simulink library "outp"  (R2021b)
(part 10 of 10)

  VTPM_LRWheelDebug_flg/1 -> VTPM_LRWheelDebug_flg_Inproc/1  "VTPM_LRWheelDebug_flg"
  VTPM_LRWheelDebug_flg_Inproc/1 -> UnitConverter666/1
  UnitConverter666/1 -> VOUTP_LRWheelDebug_flg/1  "VOUTP_LRWheelDebug_flg"
  VTPM_RFWheelDebug_flg/1 -> VTPM_RFWheelDebug_flg_Inproc/1  "VTPM_RFWheelDebug_flg"
  VTPM_RFWheelDebug_flg_Inproc/1 -> UnitConverter667/1
  UnitConverter667/1 -> VOUTP_RFWheelDebug_flg/1  "VOUTP_RFWheelDebug_flg"
  VTPM_RRWheelDebug_flg/1 -> VTPM_RRWheelDebug_flg_Inproc/1  "VTPM_RRWheelDebug_flg"
  VTPM_RRWheelDebug_flg_Inproc/1 -> UnitConverter668/1
  UnitConverter668/1 -> VOUTP_RRWheelDebug_flg/1  "VOUTP_RRWheelDebug_flg"
  VTPM_TPMSResButtAllow_flg/1 -> VTPM_TPMSResButtAllow_flg_Inproc/1  "VTPM_TPMSResButtAllow_flg"
  VTPM_TPMSResButtAllow_flg_Inproc/1 -> UnitConverter669/1
  UnitConverter669/1 -> VOUTP_TPMSResButtAllow_flg/1  "VOUTP_TPMSResButtAllow_flg"
  VTPM_TPMSCaliButtAllow_flg/1 -> VTPM_TPMSCaliButtAllow_flg_Inproc/1  "VTPM_TPMSCaliButtAllow_flg"
  VTPM_TPMSCaliButtAllow_flg_Inproc/1 -> UnitConverter670/1
  UnitConverter670/1 -> VOUTP_TPMSCaliButtAllow_flg/1  "VOUTP_TPMSCaliButtAllow_flg"
  VTPM_LFPressIndi_enum/1 -> VTPM_LFPressIndi_enum_Inproc/1  "VTPM_LFPressIndi_enum"
  VTPM_LFPressIndi_enum_Inproc/1 -> UnitConverter671/1
  UnitConverter671/1 -> VOUTP_LFPressIndi_enum/1  "VOUTP_LFPressIndi_enum"
  VTPM_RFPressIndi_enum/1 -> VTPM_RFPressIndi_enum_Inproc/1  "VTPM_RFPressIndi_enum"
  VTPM_RFPressIndi_enum_Inproc/1 -> UnitConverter672/1
  UnitConverter672/1 -> VOUTP_RFPressIndi_enum/1  "VOUTP_RFPressIndi_enum"
  VTPM_LRPressIndi_enum/1 -> VTPM_LRPressIndi_enum_Inproc/1  "VTPM_LRPressIndi_enum"
  VTPM_LRPressIndi_enum_Inproc/1 -> UnitConverter673/1
  UnitConverter673/1 -> VOUTP_LRPressIndi_enum/1  "VOUTP_LRPressIndi_enum"
  VTPM_RRPressIndi_enum/1 -> VTPM_RRPressIndi_enum_Inproc/1  "VTPM_RRPressIndi_enum"
  VTPM_RRPressIndi_enum_Inproc/1 -> UnitConverter674/1
  UnitConverter674/1 -> VOUTP_RRPressIndi_enum/1  "VOUTP_RRPressIndi_enum"
  VTPM_TPMSWarnIndi_enum/1 -> VTPM_TPMSWarnIndi_enum_Inproc/1  "VTPM_TPMSWarnIndi_enum"
  VTPM_TPMSWarnIndi_enum_Inproc/1 -> UnitConverter675/1
  UnitConverter675/1 -> VOUTP_TPMSWarnIndi_enum/1  "VOUTP_TPMSWarnIndi_enum"
  VTPM_LFWheelTmpIndi_flg/1 -> VTPM_LFWheelTmpIndi_flg_Inproc/1  "VTPM_LFWheelTmpIndi_flg"
  VTPM_LFWheelTmpIndi_flg_Inproc/1 -> UnitConverter676/1
  UnitConverter676/1 -> VOUTP_LFWheelTmpIndi_flg/1  "VOUTP_LFWheelTmpIndi_flg"
  VTPM_RFWheelTmpIndi_flg/1 -> VTPM_RFWheelTmpIndi_flg_Inproc/1  "VTPM_RFWheelTmpIndi_flg"
  VTPM_RFWheelTmpIndi_flg_Inproc/1 -> UnitConverter677/1
  UnitConverter677/1 -> VOUTP_RFWheelTmpIndi_flg/1  "VOUTP_RFWheelTmpIndi_flg"
  VTPM_LRWheelTmpIndi_flg/1 -> VTPM_LRWheelTmpIndi_flg_Inproc/1  "VTPM_LRWheelTmpIndi_flg"
  VTPM_LRWheelTmpIndi_flg_Inproc/1 -> UnitConverter678/1
  UnitConverter678/1 -> VOUTP_LRWheelTmpIndi_flg/1  "VOUTP_LRWheelTmpIndi_flg"
  VTPM_RRWheelTmpIndi_flg/1 -> VTPM_RRWheelTmpIndi_flg_Inproc/1  "VTPM_RRWheelTmpIndi_flg"
  VTPM_RRWheelTmpIndi_flg_Inproc/1 -> UnitConverter679/1
  UnitConverter679/1 -> VOUTP_RRWheelTmpIndi_flg/1  "VOUTP_RRWheelTmpIndi_flg"
  VTPM_LFWheelPSW_raw8/1 -> VTPM_LFWheelPSW_raw8_Inproc/1  "VTPM_LFWheelPSW_raw8"
  VTPM_LFWheelPSW_raw8_Inproc/1 -> UnitConverter680/1
  UnitConverter680/1 -> VOUTP_LFWheelPSW_raw8/1  "VOUTP_LFWheelPSW_raw8"
  VTPM_LRWheelPSW_raw8/1 -> VTPM_LRWheelPSW_raw8_Inproc/1  "VTPM_LRWheelPSW_raw8"
  VTPM_LRWheelPSW_raw8_Inproc/1 -> UnitConverter681/1
  UnitConverter681/1 -> VOUTP_LRWheelPSW_raw8/1  "VOUTP_LRWheelPSW_raw8"
  VTPM_RFWheelPSW_raw8/1 -> VTPM_RFWheelPSW_raw8_Inproc/1  "VTPM_RFWheelPSW_raw8"
  VTPM_RFWheelPSW_raw8_Inproc/1 -> UnitConverter682/1
  UnitConverter682/1 -> VOUTP_RFWheelPSW_raw8/1  "VOUTP_RFWheelPSW_raw8"
  VTPM_RRWheelPSW_raw8/1 -> VTPM_RRWheelPSW_raw8_Inproc/1  "VTPM_RRWheelPSW_raw8"
  VTPM_RRWheelPSW_raw8_Inproc/1 -> UnitConverter683/1
  UnitConverter683/1 -> VOUTP_RRWheelPSW_raw8/1  "VOUTP_RRWheelPSW_raw8"
  VTPM_CWheelTips_enum/1 -> VTPM_CWheelTips_enum_Inproc/1  "VTPM_CWheelTips_enum"
  VTPM_CWheelTips_enum_Inproc/1 -> UnitConverter684/1
  UnitConverter684/1 -> VOUTP_CWheelTips_enum/1  "VOUTP_CWheelTips_enum"
  VTPM_AutoLTips_enum/1 -> VTPM_AutoLTips_enum_Inproc/1  "VTPM_AutoLTips_enum"
  VTPM_AutoLTips_enum_Inproc/1 -> UnitConverter685/1
  UnitConverter685/1 -> VOUTP_AutoLTips_enum/1  "VOUTP_AutoLTips_enum"
  VTPM_LFSensorMode_flg/1 -> VTPM_LFSensorMode_flg_Inproc/1  "VTPM_LFSensorMode_flg"
  VTPM_LFSensorMode_flg_Inproc/1 -> UnitConverter686/1
  UnitConverter686/1 -> VOUTP_LFSensorMode_flg/1  "VOUTP_LFSensorMode_flg"
  VTPM_RFSensorMode_flg/1 -> VTPM_RFSensorMode_flg_Inproc/1  "VTPM_RFSensorMode_flg"
  VTPM_RFSensorMode_flg_Inproc/1 -> UnitConverter687/1
  UnitConverter687/1 -> VOUTP_RFSensorMode_flg/1  "VOUTP_RFSensorMode_flg"
  VTPM_LRSensorMode_flg/1 -> VTPM_LRSensorMode_flg_Inproc/1  "VTPM_LRSensorMode_flg"
  VTPM_LRSensorMode_flg_Inproc/1 -> UnitConverter688/1
  UnitConverter688/1 -> VOUTP_LRSensorMode_flg/1  "VOUTP_LRSensorMode_flg"
  VTPM_RRSensorMode_flg/1 -> VTPM_RRSensorMode_flg_Inproc/1  "VTPM_RRSensorMode_flg"
  VTPM_RRSensorMode_flg_Inproc/1 -> UnitConverter689/1
  UnitConverter689/1 -> VOUTP_RRSensorMode_flg/1  "VOUTP_RRSensorMode_flg"
  VTPM_S1ID_raw32/1 -> VTPM_S1ID_raw32_Inproc/1  "VTPM_S1ID_raw32"
  VTPM_S1ID_raw32_Inproc/1 -> UnitConverter690/1
  UnitConverter690/1 -> VOUTP_S1ID_raw32/1  "VOUTP_S1ID_raw32"
  VTPM_S2ID_raw32/1 -> VTPM_S2ID_raw32_Inproc/1  "VTPM_S2ID_raw32"
  VTPM_S2ID_raw32_Inproc/1 -> UnitConverter691/1
  UnitConverter691/1 -> VOUTP_S2ID_raw32/1  "VOUTP_S2ID_raw32"
  VTPM_S3ID_raw32/1 -> VTPM_S3ID_raw32_Inproc/1  "VTPM_S3ID_raw32"
  VTPM_S3ID_raw32_Inproc/1 -> UnitConverter692/1
  UnitConverter692/1 -> VOUTP_S3ID_raw32/1  "VOUTP_S3ID_raw32"
  VTPM_S4ID_raw32/1 -> VTPM_S4ID_raw32_Inproc/1  "VTPM_S4ID_raw32"
  VTPM_S4ID_raw32_Inproc/1 -> UnitConverter693/1
  UnitConverter693/1 -> VOUTP_S4ID_raw32/1  "VOUTP_S4ID_raw32"
  VTPM_S1L_enum/1 -> VTPM_S1L_enum_Inproc/1  "VTPM_S1L_enum"
  VTPM_S1L_enum_Inproc/1 -> UnitConverter694/1
  UnitConverter694/1 -> VOUTP_S1L_enum/1  "VOUTP_S1L_enum"
  VTPM_S2L_enum/1 -> VTPM_S2L_enum_Inproc/1  "VTPM_S2L_enum"
  VTPM_S2L_enum_Inproc/1 -> UnitConverter695/1
  UnitConverter695/1 -> VOUTP_S2L_enum/1  "VOUTP_S2L_enum"
  VTPM_S3L_enum/1 -> VTPM_S3L_enum_Inproc/1  "VTPM_S3L_enum"
  VTPM_S3L_enum_Inproc/1 -> UnitConverter696/1
  UnitConverter696/1 -> VOUTP_S3L_enum/1  "VOUTP_S3L_enum"
  VTPM_S4L_enum/1 -> VTPM_S4L_enum_Inproc/1  "VTPM_S4L_enum"
  VTPM_S4L_enum_Inproc/1 -> UnitConverter697/1
  UnitConverter697/1 -> VOUTP_S4L_enum/1  "VOUTP_S4L_enum"
  VTPM_ALFin_flg/1 -> VTPM_ALFin_flg_Inproc/1  "VTPM_ALFin_flg"
  VTPM_ALFin_flg_Inproc/1 -> UnitConverter698/1
  UnitConverter698/1 -> VOUTP_ALFin_flg/1  "VOUTP_ALFin_flg"
  VTPM_LFP20_raw8/1 -> VTPM_LFP20_raw8_Inproc/1  "VTPM_LFP20_raw8"
  VTPM_LFP20_raw8_Inproc/1 -> UnitConverter699/1
  UnitConverter699/1 -> VOUTP_LFP20_raw8/1  "VOUTP_LFP20_raw8"
  VTPM_RFP20_raw8/1 -> VTPM_RFP20_raw8_Inproc/1  "VTPM_RFP20_raw8"
  VTPM_RFP20_raw8_Inproc/1 -> UnitConverter700/1
  UnitConverter700/1 -> VOUTP_RFP20_raw8/1  "VOUTP_RFP20_raw8"
  VTPM_LRP20_raw8/1 -> VTPM_LRP20_raw8_Inproc/1  "VTPM_LRP20_raw8"
  VTPM_LRP20_raw8_Inproc/1 -> UnitConverter701/1
  UnitConverter701/1 -> VOUTP_LRP20_raw8/1  "VOUTP_LRP20_raw8"
  VTPM_RRP20_raw8/1 -> VTPM_RRP20_raw8_Inproc/1  "VTPM_RRP20_raw8"
  VTPM_RRP20_raw8_Inproc/1 -> UnitConverter702/1
  UnitConverter702/1 -> VOUTP_RRP20_raw8/1  "VOUTP_RRP20_raw8"
  VTPM_FAT_flg/1 -> VTPM_FAT_flg_Inproc/1  "VTPM_FAT_flg"
  VTPM_FAT_flg_Inproc/1 -> UnitConverter703/1
  UnitConverter703/1 -> VOUTP_FAT_flg/1  "VOUTP_FAT_flg"
  VTPM_IDin_raw32/1 -> VTPM_IDin_raw32_Inproc/1  "VTPM_IDin_raw32"
  VTPM_IDin_raw32_Inproc/1 -> UnitConverter704/1
  UnitConverter704/1 -> VOUTP_IDin_raw32/1  "VOUTP_IDin_raw32"
  VTPM_S1WheelDebugALTU_pct/1 -> VTPM_S1WheelDebugALTU_pct_Inproc/1  "VTPM_S1WheelDebugALTU_pct"
  VTPM_S1WheelDebugALTU_pct_Inproc/1 -> UnitConverter705/1
  UnitConverter705/1 -> VOUTP_S1WheelDebugALTU_pct/1  "VOUTP_S1WheelDebugALTU_pct"
  VTPM_S2WheelDebugALTU_pct/1 -> VTPM_S2WheelDebugALTU_pct_Inproc/1  "VTPM_S2WheelDebugALTU_pct"
  VTPM_S2WheelDebugALTU_pct_Inproc/1 -> UnitConverter706/1
  UnitConverter706/1 -> VOUTP_S2WheelDebugALTU_pct/1  "VOUTP_S2WheelDebugALTU_pct"
  VTPM_S3WheelDebugALTU_pct/1 -> VTPM_S3WheelDebugALTU_pct_Inproc/1  "VTPM_S3WheelDebugALTU_pct"
  VTPM_S3WheelDebugALTU_pct_Inproc/1 -> UnitConverter707/1
  UnitConverter707/1 -> VOUTP_S3WheelDebugALTU_pct/1  "VOUTP_S3WheelDebugALTU_pct"
  VTPM_S4WheelDebugALTU_pct/1 -> VTPM_S4WheelDebugALTU_pct_Inproc/1  "VTPM_S4WheelDebugALTU_pct"
  VTPM_S4WheelDebugALTU_pct_Inproc/1 -> UnitConverter708/1
  UnitConverter708/1 -> VOUTP_S4WheelDebugALTU_pct/1  "VOUTP_S4WheelDebugALTU_pct"
  VTPM_ID1messageALTU_raw8/1 -> VTPM_ID1messageALTU_raw8_Inproc/1  "VTPM_ID1messageALTU_raw8"
  VTPM_ID1messageALTU_raw8_Inproc/1 -> UnitConverter709/1
  UnitConverter709/1 -> VOUTP_ID1messageALTU_raw8/1  "VOUTP_ID1messageALTU_raw8"
  VTPM_ID2messageALTU_raw8/1 -> VTPM_ID2messageALTU_raw8_Inproc/1  "VTPM_ID2messageALTU_raw8"
  VTPM_ID2messageALTU_raw8_Inproc/1 -> UnitConverter710/1
  UnitConverter710/1 -> VOUTP_ID2messageALTU_raw8/1  "VOUTP_ID2messageALTU_raw8"
  VTPM_ID3messageALTU_raw8/1 -> VTPM_ID3messageALTU_raw8_Inproc/1  "VTPM_ID3messageALTU_raw8"
  VTPM_ID3messageALTU_raw8_Inproc/1 -> UnitConverter711/1
  UnitConverter711/1 -> VOUTP_ID3messageALTU_raw8/1  "VOUTP_ID3messageALTU_raw8"
  VTPM_ID4messageALTU_raw8/1 -> VTPM_ID4messageALTU_raw8_Inproc/1  "VTPM_ID4messageALTU_raw8"
  VTPM_ID4messageALTU_raw8_Inproc/1 -> UnitConverter712/1
  UnitConverter712/1 -> VOUTP_ID4messageALTU_raw8/1  "VOUTP_ID4messageALTU_raw8"
  VTPM_Chkfin_flg/1 -> VTPM_Chkfin_flg_Inproc/1  "VTPM_Chkfin_flg"
  VTPM_Chkfin_flg_Inproc/1 -> UnitConverter713/1
  UnitConverter713/1 -> VOUTP_Chkfin_flg/1  "VOUTP_Chkfin_flg"
  VTPM_SetIDLoc_flg/1 -> VTPM_SetIDLoc_flg_Inproc/1  "VTPM_SetIDLoc_flg"
  VTPM_SetIDLoc_flg_Inproc/1 -> UnitConverter714/1
  UnitConverter714/1 -> VOUTP_SetIDLoc_flg/1  "VOUTP_SetIDLoc_flg"
  VTPM_TPMSStorge_flg/1 -> VTPM_TPMSStorge_flg_Inproc/1  "VTPM_TPMSStorge_flg"
  VTPM_TPMSStorge_flg_Inproc/1 -> UnitConverter715/1
  UnitConverter715/1 -> VOUTP_TPMSStorge_flg/1  "VOUTP_TPMSStorge_flg"
  VTPM_ChkStorge_flg/1 -> VTPM_ChkStorge_flg_Inproc/1  "VTPM_ChkStorge_flg"
  VTPM_ChkStorge_flg_Inproc/1 -> UnitConverter716/1
  UnitConverter716/1 -> VOUTP_ChkStorge_flg/1  "VOUTP_ChkStorge_flg"
  VTPM_TPMSResButt_flg/1 -> VTPM_TPMSResButt_flg_Inproc/1  "VTPM_TPMSResButt_flg"
  VTPM_TPMSResButt_flg_Inproc/1 -> UnitConverter717/1
  UnitConverter717/1 -> VOUTP_TPMSResButt_flg/1  "VOUTP_TPMSResButt_flg"
  VTPM_LFPindi_enum/1 -> VTPM_LFPindi_enum_Inproc/1  "VTPM_LFPindi_enum"
  VTPM_LFPindi_enum_Inproc/1 -> UnitConverter718/1
  UnitConverter718/1 -> VOUTP_LFPindi_enum/1  "VOUTP_LFPindi_enum"
  VTPM_RFPind_enum/1 -> VTPM_RFPind_enum_Inproc/1  "VTPM_RFPind_enum"
  VTPM_RFPind_enum_Inproc/1 -> UnitConverter719/1
  UnitConverter719/1 -> VOUTP_RFPind_enum/1  "VOUTP_RFPind_enum"
  VTPM_LRPindi_enum/1 -> VTPM_LRPindi_enum_Inproc/1  "VTPM_LRPindi_enum"
  VTPM_LRPindi_enum_Inproc/1 -> UnitConverter720/1
  UnitConverter720/1 -> VOUTP_LRPindi_enum/1  "VOUTP_LRPindi_enum"
  VTPM_RRPindi_enum/1 -> VTPM_RRPindi_enum_Inproc/1  "VTPM_RRPindi_enum"
  VTPM_RRPindi_enum_Inproc/1 -> UnitConverter721/1
  UnitConverter721/1 -> VOUTP_RRPindi_enum/1  "VOUTP_RRPindi_enum"
  VTPM_WriteChkLFID_raw/1 -> VTPM_WriteChkLFID_raw_Inproc/1  "VTPM_WriteChkLFID_raw"
  VTPM_WriteChkLFID_raw_Inproc/1 -> UnitConverter722/1
  UnitConverter722/1 -> VOUTP_WriteChkLFID_raw/1  "VOUTP_WriteChkLFID_raw"
  VTPM_WriteChkRFID_raw/1 -> VTPM_WriteChkRFID_raw_Inproc/1  "VTPM_WriteChkRFID_raw"
  VTPM_WriteChkRFID_raw_Inproc/1 -> UnitConverter723/1
  UnitConverter723/1 -> VOUTP_WriteChkRFID_raw/1  "VOUTP_WriteChkRFID_raw"
  VTPM_WriteChkLRID_raw/1 -> VTPM_WriteChkLRID_raw_Inproc/1  "VTPM_WriteChkLRID_raw"
  VTPM_WriteChkLRID_raw_Inproc/1 -> UnitConverter724/1
  UnitConverter724/1 -> VOUTP_WriteChkLRID_raw/1  "VOUTP_WriteChkLRID_raw"
  VTPM_WriteChkRRID_raw/1 -> VTPM_WriteChkRRID_raw_Inproc/1  "VTPM_WriteChkRRID_raw"
  VTPM_WriteChkRRID_raw_Inproc/1 -> UnitConverter725/1
  UnitConverter725/1 -> VOUTP_WriteChkRRID_raw/1  "VOUTP_WriteChkRRID_raw"
  VTPM_WriteChkfinLFID_raw/1 -> VTPM_WriteChkfinLFID_raw_Inproc/1  "VTPM_WriteChkfinLFID_raw"
  VTPM_WriteChkfinLFID_raw_Inproc/1 -> UnitConverter726/1
  UnitConverter726/1 -> VOUTP_WriteChkfinLFID_raw/1  "VOUTP_WriteChkfinLFID_raw"
  VTPM_WriteChkfinRFID_raw/1 -> VTPM_WriteChkfinRFID_raw_Inproc/1  "VTPM_WriteChkfinRFID_raw"
  VTPM_WriteChkfinRFID_raw_Inproc/1 -> UnitConverter727/1
  UnitConverter727/1 -> VOUTP_WriteChkfinRFID_raw/1  "VOUTP_WriteChkfinRFID_raw"
  VTPM_WriteChkfinLRID_raw/1 -> VTPM_WriteChkfinLRID_raw_Inproc/1  "VTPM_WriteChkfinLRID_raw"
  VTPM_WriteChkfinLRID_raw_Inproc/1 -> UnitConverter728/1
  UnitConverter728/1 -> VOUTP_WriteChkfinLRID_raw/1  "VOUTP_WriteChkfinLRID_raw"
  VTPM_WriteChkfinRRID_raw/1 -> VTPM_WriteChkfinRRID_raw_Inproc/1  "VTPM_WriteChkfinRRID_raw"
  VTPM_WriteChkfinRRID_raw_Inproc/1 -> UnitConverter729/1
  UnitConverter729/1 -> VOUTP_WriteChkfinRRID_raw/1  "VOUTP_WriteChkfinRRID_raw"
  VTPM_Flashchkdatavalid_enum/1 -> VTPM_Flashchkdatavalid_enum_Inproc/1  "VTPM_Flashchkdatavalid_enum"
  VTPM_Flashchkdatavalid_enum_Inproc/1 -> UnitConverter730/1
  UnitConverter730/1 -> VOUTP_Flashchkdatavalid_enum/1  "VOUTP_Flashchkdatavalid_enum"
  VTPM_Flashdatavalid_enum/1 -> VTPM_Flashdatavalid_enum_Inproc/1  "VTPM_Flashdatavalid_enum"
  VTPM_Flashdatavalid_enum_Inproc/1 -> UnitConverter731/1
  UnitConverter731/1 -> VOUTP_Flashdatavalid_enum/1  "VOUTP_Flashdatavalid_enum"
  VTPM_unlearnSfali_flg/1 -> VTPM_unlearnSfali_flg_Inproc/1  "VTPM_unlearnSfali_flg"
  VTPM_unlearnSfali_flg_Inproc/1 -> UnitConverter732/1
  UnitConverter732/1 -> VOUTP_unlearnSfali_flg/1  "VOUTP_unlearnSfali_flg"
  VTPM_unlearnSfailvalid_enum/1 -> VTPM_unlearnSfailvalid_enum_Inproc/1  "VTPM_unlearnSfailvalid_enum"
  VTPM_unlearnSfailvalid_enum_Inproc/1 -> UnitConverter733/1
  UnitConverter733/1 -> VOUTP_unlearnSfailvalid_enum/1  "VOUTP_unlearnSfailvalid_enum"
  VTPM_Prepresstempvalid_enum/1 -> VTPM_Prepresstempvalid_enum_Inproc/1  "VTPM_Prepresstempvalid_enum"
  VTPM_Prepresstempvalid_enum_Inproc/1 -> UnitConverter734/1
  UnitConverter734/1 -> VOUTP_Prepresstempvalid_enum/1  "VOUTP_Prepresstempvalid_enum"
  VTPM_FlashS1ID_raw/1 -> VTPM_FlashS1ID_raw_Inproc/1  "VTPM_FlashS1ID_raw"
  VTPM_FlashS1ID_raw_Inproc/1 -> UnitConverter735/1
  UnitConverter735/1 -> VOUTP_FlashS1ID_raw/1  "VOUTP_FlashS1ID_raw"
  VTPM_FlashS2ID_raw/1 -> VTPM_FlashS2ID_raw_Inproc/1  "VTPM_FlashS2ID_raw"
  VTPM_FlashS2ID_raw_Inproc/1 -> UnitConverter736/1
  UnitConverter736/1 -> VOUTP_FlashS2ID_raw/1  "VOUTP_FlashS2ID_raw"
  VTPM_FlashS3ID_raw/1 -> VTPM_FlashS3ID_raw_Inproc/1  "VTPM_FlashS3ID_raw"
  VTPM_FlashS3ID_raw_Inproc/1 -> UnitConverter737/1
  UnitConverter737/1 -> VOUTP_FlashS3ID_raw/1  "VOUTP_FlashS3ID_raw"
  VTPM_FlashS4ID_raw/1 -> VTPM_FlashS4ID_raw_Inproc/1  "VTPM_FlashS4ID_raw"
  VTPM_FlashS4ID_raw_Inproc/1 -> UnitConverter738/1
  UnitConverter738/1 -> VOUTP_FlashS4ID_raw/1  "VOUTP_FlashS4ID_raw"
  VTPM_FlashIDvalid_enum/1 -> VTPM_FlashIDvalid_enum_Inproc/1  "VTPM_FlashIDvalid_enum"
  VTPM_FlashIDvalid_enum_Inproc/1 -> UnitConverter739/1
  UnitConverter739/1 -> VOUTP_FlashIDvalid_enum/1  "VOUTP_FlashIDvalid_enum"
  VTPM_WritingCnt_enum/1 -> VTPM_WritingCnt_enum_Inproc/1  "VTPM_WritingCnt_enum"
  VTPM_WritingCnt_enum_Inproc/1 -> UnitConverter740/1
  UnitConverter740/1 -> VOUTP_WritingCnt_enum/1  "VOUTP_WritingCnt_enum"
  VTPM_TPMSTLCmd_flg/1 -> VTPM_TPMSTLCmd_flg_Inproc/1  "VTPM_TPMSTLCmd_flg"
  VTPM_TPMSTLCmd_flg_Inproc/1 -> UnitConverter741/1
  UnitConverter741/1 -> VOUTP_TPMSTLCmd_flg/1  "VOUTP_TPMSTLCmd_flg"
  VTPM_LProgress_enum/1 -> VTPM_LProgress_enum_Inproc/1  "VTPM_LProgress_enum"
  VTPM_LProgress_enum_Inproc/1 -> UnitConverter742/1
  UnitConverter742/1 -> VOUTP_LProgress_enum/1  "VOUTP_LProgress_enum"
  VTPM_TPMSSensorIDRegStart_flg/1 -> VTPM_TPMSSensorIDRegStart_flg_Inproc/1  "VTPM_TPMSSensorIDRegStart_flg"
  VTPM_TPMSSensorIDRegStart_flg_Inproc/1 -> UnitConverter743/1
  UnitConverter743/1 -> VOUTP_TPMSSensorIDRegStart_flg/1  "VOUTP_TPMSSensorIDRegStart_flg"
  VTPM_ModelVersion_raw/1 -> VTPM_ModelVersion_raw_Inproc/1  "VTPM_ModelVersion_raw"
  VTPM_ModelVersion_raw_Inproc/1 -> UnitConverter744/1
  UnitConverter744/1 -> VOUTP_ModelVersion_raw/1  "VOUTP_ModelVersion_raw"
  VTPM_ModelVersionChksum_raw/1 -> VTPM_ModelVersionChksum_raw_Inproc/1  "VTPM_ModelVersionChksum_raw"
  VTPM_ModelVersionChksum_raw_Inproc/1 -> UnitConverter745/1
  UnitConverter745/1 -> VOUTP_ModelVersionChksum_raw/1  "VOUTP_ModelVersionChksum_raw"
  VTQD_VCUMCUCtrlMdTQD_enum/1 -> VTQD_VCUMCUCtrlMdTQD_enum_Inproc/1  "VTQD_VCUMCUCtrlMdTQD_enum"
  VTQD_VCUMCUCtrlMdTQD_enum_Inproc/1 -> UnitConverter746/1
  UnitConverter746/1 -> VOUTP_VCUMCUCtrlMdTQD_enum/1  "VOUTP_VCUMCUCtrlMdTQD_enum"
  VTQD_CreepSpdReq_rpm/1 -> VTQD_CreepSpdReq_rpm_Inproc/1  "VTQD_CreepSpdReq_rpm"
  VTQD_CreepSpdReq_rpm_Inproc/1 -> UnitConverter747/1
  UnitConverter747/1 -> VOUTP_CreepSpdReq_rpm/1  "VOUTP_CreepSpdReq_rpm"
  VTQD_CreepIND_enum/1 -> VTQD_CreepIND_enum_Inproc/1  "VTQD_CreepIND_enum"
  VTQD_CreepIND_enum_Inproc/1 -> UnitConverter748/1
  UnitConverter748/1 -> VOUTP_CreepIND_enum/1  "VOUTP_CreepIND_enum"
  VTQD_ActTUpAIND_enum/1 -> VTQD_ActTUpAIND_enum_Inproc/1  "VTQD_ActTUpAIND_enum"
  VTQD_ActTUpAIND_enum_Inproc/1 -> UnitConverter749/1
  UnitConverter749/1 -> VOUTP_ActTUpAIND_enum/1  "VOUTP_ActTUpAIND_enum"
  VTQD_VCUMCUDemHiPosVal_rpm/1 -> VTQD_VCUMCUDemHiPosVal_rpm_Inproc/1  "VTQD_VCUMCUDemHiPosVal_rpm"
  VTQD_VCUMCUDemHiPosVal_rpm_Inproc/1 -> UnitConverter750/1
  UnitConverter750/1 -> VOUTP_VCUMCUDemHiPosVal_rpm/1  "VOUTP_VCUMCUDemHiPosVal_rpm"
  VTQD_VehAcclLimitTG_mps2/1 -> VTQD_VehAcclLimitTG_mps2_Inproc/1  "VTQD_VehAcclLimitTG_mps2"
  VTQD_VehAcclLimitTG_mps2_Inproc/1 -> UnitConverter751/1
  UnitConverter751/1 -> VOUTP_VehAcclLimitTG_mps2/1  "VOUTP_VehAcclLimitTG_mps2"
  VTQD_VCUEBSHHSw_enum/1 -> VTQD_VCUEBSHHSw_enum_Inproc/1  "VTQD_VCUEBSHHSw_enum"
  VTQD_VCUEBSHHSw_enum_Inproc/1 -> UnitConverter752/1
  UnitConverter752/1 -> VOUTP_VCUEBSHHSw_enum/1  "VOUTP_VCUEBSHHSw_enum"
  VTQD_VCUEBSRd4BR_enum/1 -> VTQD_VCUEBSRd4BR_enum_Inproc/1  "VTQD_VCUEBSRd4BR_enum"
  VTQD_VCUEBSRd4BR_enum_Inproc/1 -> UnitConverter753/1
  UnitConverter753/1 -> VOUTP_VCUEBSRd4BR_enum/1  "VOUTP_VCUEBSRd4BR_enum"
  VTQD_ParkingProtectWarning_flg/1 -> VTQD_ParkingProtectWarning_flg_Inproc/1  "VTQD_ParkingProtectWarning_flg"
  VTQD_ParkingProtectWarning_flg_Inproc/1 -> UnitConverter754/1
  UnitConverter754/1 -> VOUTP_ParkingProtectWarning_flg/1  "VOUTP_ParkingProtectWarning_flg"
  VTQD_ActDriveMode_enum/1 -> VTQD_ActDriveMode_enum_Inproc/1  "VTQD_ActDriveMode_enum"
  VTQD_ActDriveMode_enum_Inproc/1 -> UnitConverter755/1
  UnitConverter755/1 -> VOUTP_ActDriveMode_enum/1  "VOUTP_ActDriveMode_enum"
  VTQD_VCU4PweLmtInd_flg/1 -> VTQD_VCU4PweLmtInd_flg_Inproc/1  "VTQD_VCU4PweLmtInd_flg"
  VTQD_VCU4PweLmtInd_flg_Inproc/1 -> UnitConverter756/1
  UnitConverter756/1 -> VOUTP_VCU4PweLmtInd_flg/1  "VOUTP_VCU4PweLmtInd_flg"
  VTQD_GearFlashIndDis_flg/1 -> VTQD_GearFlashIndDis_flg_Inproc/1  "VTQD_GearFlashIndDis_flg"
  VTQD_GearFlashIndDis_flg_Inproc/1 -> UnitConverter757/1
  UnitConverter757/1 -> VOUTP_GearFlashIndDis_flg/1  "VOUTP_GearFlashIndDis_flg"
  VTQD_GearFlashInd_flg/1 -> VTQD_GearFlashInd_flg_Inproc/1  "VTQD_GearFlashInd_flg"
  VTQD_GearFlashInd_flg_Inproc/1 -> UnitConverter758/1
  UnitConverter758/1 -> VOUTP_GearFlashInd_flg/1  "VOUTP_GearFlashInd_flg"
  VTQD_SpdLimSta_flg/1 -> VTQD_SpdLimSta_flg_Inproc/1  "VTQD_SpdLimSta_flg"
  VTQD_SpdLimSta_flg_Inproc/1 -> UnitConverter759/1
  UnitConverter759/1 -> VOUTP_SpdLimSta_flg/1  "VOUTP_SpdLimSta_flg"
  VTQD_VehSpdLimitTG_kph/1 -> VTQD_VehSpdLimitTG_kph_Inproc/1  "VTQD_VehSpdLimitTG_kph"
  VTQD_VehSpdLimitTG_kph_Inproc/1 -> UnitConverter760/1
  UnitConverter760/1 -> VOUTP_VehSpdLimitTG_kph/1  "VOUTP_VehSpdLimitTG_kph"
  VTQD_VCUTMVehSpd_kph/1 -> VTQD_VCUTMVehSpd_kph_Inproc/1  "VTQD_VCUTMVehSpd_kph"
  VTQD_VCUTMVehSpd_kph_Inproc/1 -> UnitConverter761/1
  UnitConverter761/1 -> VOUTP_VCUTMVehSpd_kph/1  "VOUTP_VCUTMVehSpd_kph"
  VTQD_TMTqReq_Nm/1 -> VTQD_TMTqReq_Nm_Inproc/1  "VTQD_TMTqReq_Nm"
  VTQD_TMTqReq_Nm_Inproc/1 -> UnitConverter762/1
  UnitConverter762/1 -> VOUTP_TMTqReq_Nm/1  "VOUTP_TMTqReq_Nm"
  VTQD_VCUBCMBuzzReq_flg/1 -> VTQD_VCUBCMBuzzReq_flg_Inproc/1  "VTQD_VCUBCMBuzzReq_flg"
  VTQD_VCUBCMBuzzReq_flg_Inproc/1 -> UnitConverter763/1
  UnitConverter763/1 -> VOUTP_VCUBCMBuzzReq_flg/1  "VOUTP_VCUBCMBuzzReq_flg"
  VTQD_VCUEBSHBSw_enum/1 -> VTQD_VCUEBSHBSw_enum_Inproc/1  "VTQD_VCUEBSHBSw_enum"
  VTQD_VCUEBSHBSw_enum_Inproc/1 -> UnitConverter764/1
  UnitConverter764/1 -> VOUTP_VCUEBSHBSw_enum/1  "VOUTP_VCUEBSHBSw_enum"
  VTQD_EVCU1ActDrvMode_enum/1 -> VTQD_EVCU1ActDrvMode_enum_Inproc/1  "VTQD_EVCU1ActDrvMode_enum"
  VTQD_EVCU1ActDrvMode_enum_Inproc/1 -> UnitConverter765/1
  UnitConverter765/1 -> VOUTP_EVCU1ActDrvMode_enum/1  "VOUTP_EVCU1ActDrvMode_enum"
  VTQD_EVCU1WheelSlipdet_enum/1 -> VTQD_EVCU1WheelSlipdet_enum_Inproc/1  "VTQD_EVCU1WheelSlipdet_enum"
  VTQD_EVCU1WheelSlipdet_enum_Inproc/1 -> UnitConverter766/1
  UnitConverter766/1 -> VOUTP_EVCU1WheelSlipdet_enum/1  "VOUTP_EVCU1WheelSlipdet_enum"
  VTQD_EVCU1EMotorSpd_rpm/1 -> VTQD_EVCU1EMotorSpd_rpm_Inproc/1  "VTQD_EVCU1EMotorSpd_rpm"
  VTQD_EVCU1EMotorSpd_rpm_Inproc/1 -> UnitConverter767/1
  UnitConverter767/1 -> VOUTP_EVCU1EMotorSpd_rpm/1  "VOUTP_EVCU1EMotorSpd_rpm"
  VTQD_EVCU1EMotorOvrerSpd_enum/1 -> VTQD_EVCU1EMotorOvrerSpd_enum_Inproc/1  "VTQD_EVCU1EMotorOvrerSpd_enum"
  VTQD_EVCU1EMotorOvrerSpd_enum_Inproc/1 -> UnitConverter768/1
  UnitConverter768/1 -> VOUTP_EVCU1EMotorOvrerSpd_enum/1  "VOUTP_EVCU1EMotorOvrerSpd_enum"
  VTQD_EVCU1EMotorPerformance_pct/1 -> VTQD_EVCU1EMotorPerformance_pct_Inproc/1  "VTQD_EVCU1EMotorPerformance_pct"
  VTQD_EVCU1EMotorPerformance_pct_Inproc/1 -> UnitConverter769/1
  UnitConverter769/1 -> VOUTP_EVCU1EMotorPerformance_pct/1  "VOUTP_EVCU1EMotorPerformance_pct"
  VTQD_EVCU1EBrakeTorqLow_enum/1 -> VTQD_EVCU1EBrakeTorqLow_enum_Inproc/1  "VTQD_EVCU1EBrakeTorqLow_enum"
  VTQD_EVCU1EBrakeTorqLow_enum_Inproc/1 -> UnitConverter770/1
  UnitConverter770/1 -> VOUTP_EVCU1EBrakeTorqLow_enum/1  "VOUTP_EVCU1EBrakeTorqLow_enum"
  VTQD_EVCU2MaxTorqAvail_pct/1 -> VTQD_EVCU2MaxTorqAvail_pct_Inproc/1  "VTQD_EVCU2MaxTorqAvail_pct"
  VTQD_EVCU2MaxTorqAvail_pct_Inproc/1 -> UnitConverter771/1
  UnitConverter771/1 -> VOUTP_EVCU2MaxTorqAvail_pct/1  "VOUTP_EVCU2MaxTorqAvail_pct"
  VTQD_EVCU2MinTorqAvail_pct/1 -> VTQD_EVCU2MinTorqAvail_pct_Inproc/1  "VTQD_EVCU2MinTorqAvail_pct"
  VTQD_EVCU2MinTorqAvail_pct_Inproc/1 -> UnitConverter772/1
  UnitConverter772/1 -> VOUTP_EVCU2MinTorqAvail_pct/1  "VOUTP_EVCU2MinTorqAvail_pct"
  VTQD_EEC3NFricPercTorq_pct/1 -> VTQD_EEC3NFricPercTorq_pct_Inproc/1  "VTQD_EEC3NFricPercTorq_pct"
  VTQD_EEC3NFricPercTorq_pct_Inproc/1 -> UnitConverter773/1
  UnitConverter773/1 -> VOUTP_EEC3NFricPercTorq_pct/1  "VOUTP_EEC3NFricPercTorq_pct"
  VTQD_EEC3EMPressLoss_pct/1 -> VTQD_EEC3EMPressLoss_pct_Inproc/1  "VTQD_EEC3EMPressLoss_pct"
  VTQD_EEC3EMPressLoss_pct_Inproc/1 -> UnitConverter774/1
  UnitConverter774/1 -> VOUTP_EEC3EMPressLoss_pct/1  "VOUTP_EEC3EMPressLoss_pct"
  VTQD_ETC2ActDriveDirect_enum/1 -> VTQD_ETC2ActDriveDirect_enum_Inproc/1  "VTQD_ETC2ActDriveDirect_enum"
  VTQD_ETC2ActDriveDirect_enum_Inproc/1 -> UnitConverter775/1
  UnitConverter775/1 -> VOUTP_ETC2ActDriveDirect_enum/1  "VOUTP_ETC2ActDriveDirect_enum"
  VTQD_RC1PctTrqP4_pct/1 -> VTQD_RC1PctTrqP4_pct_Inproc/1  "VTQD_RC1PctTrqP4_pct"
  VTQD_RC1PctTrqP4_pct_Inproc/1 -> UnitConverter776/1
  UnitConverter776/1 -> VOUTP_RC1PctTrqP4_pct/1  "VOUTP_RC1PctTrqP4_pct"
  VTQD_RC1PctTrqPekTrqP5_pct/1 -> VTQD_RC1PctTrqPekTrqP5_pct_Inproc/1  "VTQD_RC1PctTrqPekTrqP5_pct"
  VTQD_RC1PctTrqPekTrqP5_pct_Inproc/1 -> UnitConverter777/1
  UnitConverter777/1 -> VOUTP_RC1PctTrqPekTrqP5_pct/1  "VOUTP_RC1PctTrqPekTrqP5_pct"
  VTQD_EMRC1EMTquModeDrvBrk_enum/1 -> VTQD_EMRC1EMTquModeDrvBrk_enum_Inproc/1  "VTQD_EMRC1EMTquModeDrvBrk_enum"
  VTQD_EMRC1EMTquModeDrvBrk_enum_Inproc/1 -> UnitConverter778/1
  UnitConverter778/1 -> VOUTP_EMRC1EMTquModeDrvBrk_enum/1  "VOUTP_EMRC1EMTquModeDrvBrk_enum"
  VTQD_EMRC1ActEMpTrq_pct/1 -> VTQD_EMRC1ActEMpTrq_pct_Inproc/1  "VTQD_EMRC1ActEMpTrq_pct"
  VTQD_EMRC1ActEMpTrq_pct_Inproc/1 -> UnitConverter779/1
  UnitConverter779/1 -> VOUTP_EMRC1ActEMpTrq_pct/1  "VOUTP_EMRC1ActEMpTrq_pct"
  VTQD_EMRC1ActEMOutSftSpd_rpm/1 -> VTQD_EMRC1ActEMOutSftSpd_rpm_Inproc/1  "VTQD_EMRC1ActEMOutSftSpd_rpm"
  VTQD_EMRC1ActEMOutSftSpd_rpm_Inproc/1 -> UnitConverter780/1
  UnitConverter780/1 -> VOUTP_EMRC1ActEMOutSftSpd_rpm/1  "VOUTP_EMRC1ActEMOutSftSpd_rpm"
  VTQD_EMRC1ActEMpTrqHrls_pct/1 -> VTQD_EMRC1ActEMpTrqHrls_pct_Inproc/1  "VTQD_EMRC1ActEMpTrqHrls_pct"
  VTQD_EMRC1ActEMpTrqHrls_pct_Inproc/1 -> UnitConverter781/1
  UnitConverter781/1 -> VOUTP_EMRC1ActEMpTrqHrls_pct/1  "VOUTP_EMRC1ActEMpTrqHrls_pct"
  VTQD_EMRC1ActMaxAvaEMRecpTrq_pct/1 -> VTQD_EMRC1ActMaxAvaEMRecpTrq_pct_Inproc/1  "VTQD_EMRC1ActMaxAvaEMRecpTrq_pct"
  VTQD_EMRC1ActMaxAvaEMRecpTrq_pct_Inproc/1 -> UnitConverter782/1
  UnitConverter782/1 -> VOUTP_EMRC1ActMaxAvaEMRecpTrq_pct/1  "VOUTP_EMRC1ActMaxAvaEMRecpTrq_pct"
  VTQD_EC1EMSpdIdleP1_rpm/1 -> VTQD_EC1EMSpdIdleP1_rpm_Inproc/1  "VTQD_EC1EMSpdIdleP1_rpm"
  VTQD_EC1EMSpdIdleP1_rpm_Inproc/1 -> UnitConverter783/1
  UnitConverter783/1 -> VOUTP_EC1EMSpdIdleP1_rpm/1  "VOUTP_EC1EMSpdIdleP1_rpm"
  VTQD_EC1PercTorqIdleP1_pct/1 -> VTQD_EC1PercTorqIdleP1_pct_Inproc/1  "VTQD_EC1PercTorqIdleP1_pct"
  VTQD_EC1PercTorqIdleP1_pct_Inproc/1 -> UnitConverter784/1
  UnitConverter784/1 -> VOUTP_EC1PercTorqIdleP1_pct/1  "VOUTP_EC1PercTorqIdleP1_pct"
  VTQD_EC1EMSpdIdleP2_rpm/1 -> VTQD_EC1EMSpdIdleP2_rpm_Inproc/1  "VTQD_EC1EMSpdIdleP2_rpm"
  VTQD_EC1EMSpdIdleP2_rpm_Inproc/1 -> UnitConverter785/1
  UnitConverter785/1 -> VOUTP_EC1EMSpdIdleP2_rpm/1  "VOUTP_EC1EMSpdIdleP2_rpm"
  VTQD_EC1PercTorqIdleP2_pct/1 -> VTQD_EC1PercTorqIdleP2_pct_Inproc/1  "VTQD_EC1PercTorqIdleP2_pct"
  VTQD_EC1PercTorqIdleP2_pct_Inproc/1 -> UnitConverter786/1
  UnitConverter786/1 -> VOUTP_EC1PercTorqIdleP2_pct/1  "VOUTP_EC1PercTorqIdleP2_pct"
  VTQD_EC1EMSpdIdleP3_rpm/1 -> VTQD_EC1EMSpdIdleP3_rpm_Inproc/1  "VTQD_EC1EMSpdIdleP3_rpm"
  VTQD_EC1EMSpdIdleP3_rpm_Inproc/1 -> UnitConverter787/1
  UnitConverter787/1 -> VOUTP_EC1EMSpdIdleP3_rpm/1  "VOUTP_EC1EMSpdIdleP3_rpm"
  VTQD_EC1PercTorqIdleP3_pct/1 -> VTQD_EC1PercTorqIdleP3_pct_Inproc/1  "VTQD_EC1PercTorqIdleP3_pct"
  VTQD_EC1PercTorqIdleP3_pct_Inproc/1 -> UnitConverter788/1
  UnitConverter788/1 -> VOUTP_EC1PercTorqIdleP3_pct/1  "VOUTP_EC1PercTorqIdleP3_pct"
  VTQD_EC1EMSpdIdleP4_rpm/1 -> VTQD_EC1EMSpdIdleP4_rpm_Inproc/1  "VTQD_EC1EMSpdIdleP4_rpm"
  VTQD_EC1EMSpdIdleP4_rpm_Inproc/1 -> UnitConverter789/1
  UnitConverter789/1 -> VOUTP_EC1EMSpdIdleP4_rpm/1  "VOUTP_EC1EMSpdIdleP4_rpm"
  VTQD_EC1PercTorqIdleP4_pct/1 -> VTQD_EC1PercTorqIdleP4_pct_Inproc/1  "VTQD_EC1PercTorqIdleP4_pct"
  VTQD_EC1PercTorqIdleP4_pct_Inproc/1 -> UnitConverter790/1
  UnitConverter790/1 -> VOUTP_EC1PercTorqIdleP4_pct/1  "VOUTP_EC1PercTorqIdleP4_pct"
  VTQD_EC1PercTorqIdleP5_pct/1 -> VTQD_EC1PercTorqIdleP5_pct_Inproc/1  "VTQD_EC1PercTorqIdleP5_pct"
  VTQD_EC1PercTorqIdleP5_pct_Inproc/1 -> UnitConverter791/1
  UnitConverter791/1 -> VOUTP_EC1PercTorqIdleP5_pct/1  "VOUTP_EC1PercTorqIdleP5_pct"
  VTQD_EC1EMSpdIdleP5_rpm/1 -> VTQD_EC1EMSpdIdleP5_rpm_Inproc/1  "VTQD_EC1EMSpdIdleP5_rpm"
  VTQD_EC1EMSpdIdleP5_rpm_Inproc/1 -> UnitConverter792/1
  UnitConverter792/1 -> VOUTP_EC1EMSpdIdleP5_rpm/1  "VOUTP_EC1EMSpdIdleP5_rpm"
  VTQD_EC1EMRefTorq_Nm/1 -> VTQD_EC1EMRefTorq_Nm_Inproc/1  "VTQD_EC1EMRefTorq_Nm"
  VTQD_EC1EMRefTorq_Nm_Inproc/1 -> UnitConverter793/1
  UnitConverter793/1 -> VOUTP_EC1EMRefTorq_Nm/1  "VOUTP_EC1EMRefTorq_Nm"
  VTQD_EC1EMMaxMEngOvrSP7_rpm/1 -> VTQD_EC1EMMaxMEngOvrSP7_rpm_Inproc/1  "VTQD_EC1EMMaxMEngOvrSP7_rpm"
  VTQD_EC1EMMaxMEngOvrSP7_rpm_Inproc/1 -> UnitConverter794/1
  UnitConverter794/1 -> VOUTP_EC1EMMaxMEngOvrSP7_rpm/1  "VOUTP_EC1EMMaxMEngOvrSP7_rpm"
  VTQD_EC1EMMaxMOvrTmt_s/1 -> VTQD_EC1EMMaxMOvrTmt_s_Inproc/1  "VTQD_EC1EMMaxMOvrTmt_s"
  VTQD_EC1EMMaxMOvrTmt_s_Inproc/1 -> UnitConverter795/1
  UnitConverter795/1 -> VOUTP_EC1EMMaxMOvrTmt_s/1  "VOUTP_EC1EMMaxMOvrTmt_s"
  VTQD_EC1EMReqSpdCtrlLoLmt_rpm/1 -> VTQD_EC1EMReqSpdCtrlLoLmt_rpm_Inproc/1  "VTQD_EC1EMReqSpdCtrlLoLmt_rpm"
  VTQD_EC1EMReqSpdCtrlLoLmt_rpm_Inproc/1 -> UnitConverter796/1
  UnitConverter796/1 -> VOUTP_EC1EMReqSpdCtrlLoLmt_rpm/1  "VOUTP_EC1EMReqSpdCtrlLoLmt_rpm"
  VTQD_EC1EMReqTrqCtrlLoLmt_pct/1 -> VTQD_EC1EMReqTrqCtrlLoLmt_pct_Inproc/1  "VTQD_EC1EMReqTrqCtrlLoLmt_pct"
  VTQD_EC1EMReqTrqCtrlLoLmt_pct_Inproc/1 -> UnitConverter797/1
  UnitConverter797/1 -> VOUTP_EC1EMReqTrqCtrlLoLmt_pct/1  "VOUTP_EC1EMReqTrqCtrlLoLmt_pct"
  VTQD_EC1EMReqSpdCtrlUpLmt_rpm/1 -> VTQD_EC1EMReqSpdCtrlUpLmt_rpm_Inproc/1  "VTQD_EC1EMReqSpdCtrlUpLmt_rpm"
  VTQD_EC1EMReqSpdCtrlUpLmt_rpm_Inproc/1 -> UnitConverter798/1
  UnitConverter798/1 -> VOUTP_EC1EMReqSpdCtrlUpLmt_rpm/1  "VOUTP_EC1EMReqSpdCtrlUpLmt_rpm"
  VTQD_EC1EMReqTrqCtrlUpLmt_pct/1 -> VTQD_EC1EMReqTrqCtrlUpLmt_pct_Inproc/1  "VTQD_EC1EMReqTrqCtrlUpLmt_pct"
  VTQD_EC1EMReqTrqCtrlUpLmt_pct_Inproc/1 -> UnitConverter799/1
  UnitConverter799/1 -> VOUTP_EC1EMReqTrqCtrlUpLmt_pct/1  "VOUTP_EC1EMReqTrqCtrlUpLmt_pct"
  VTQD_EC1EMExtRSCtrlUpLmt_rpm/1 -> VTQD_EC1EMExtRSCtrlUpLmt_rpm_Inproc/1  "VTQD_EC1EMExtRSCtrlUpLmt_rpm"
  VTQD_EC1EMExtRSCtrlUpLmt_rpm_Inproc/1 -> UnitConverter800/1
  UnitConverter800/1 -> VOUTP_EC1EMExtRSCtrlUpLmt_rpm/1  "VOUTP_EC1EMExtRSCtrlUpLmt_rpm"
  VTQD_EC1EMMomOfInertia_kgpm2/1 -> VTQD_EC1EMMomOfInertia_kgpm2_Inproc/1  "VTQD_EC1EMMomOfInertia_kgpm2"
  VTQD_EC1EMMomOfInertia_kgpm2_Inproc/1 -> UnitConverter801/1
  UnitConverter801/1 -> VOUTP_EC1EMMomOfInertia_kgpm2/1  "VOUTP_EC1EMMomOfInertia_kgpm2"
  VTQD_EC1EMDefTrqLmt_rpm/1 -> VTQD_EC1EMDefTrqLmt_rpm_Inproc/1  "VTQD_EC1EMDefTrqLmt_rpm"
  VTQD_EC1EMDefTrqLmt_rpm_Inproc/1 -> UnitConverter802/1
  UnitConverter802/1 -> VOUTP_EC1EMDefTrqLmt_rpm/1  "VOUTP_EC1EMDefTrqLmt_rpm"
  VTQD_EC1EMSupVarRTSC1MSG_cnt/1 -> VTQD_EC1EMSupVarRTSC1MSG_cnt_Inproc/1  "VTQD_EC1EMSupVarRTSC1MSG_cnt"
  VTQD_EC1EMSupVarRTSC1MSG_cnt_Inproc/1 -> UnitConverter803/1
  UnitConverter803/1 -> VOUTP_EC1EMSupVarRTSC1MSG_cnt/1  "VOUTP_EC1EMSupVarRTSC1MSG_cnt"
  VTQD_EC1EMSupTSC1CtrlPG1_cnt/1 -> VTQD_EC1EMSupTSC1CtrlPG1_cnt_Inproc/1  "VTQD_EC1EMSupTSC1CtrlPG1_cnt"
  VTQD_EC1EMSupTSC1CtrlPG1_cnt_Inproc/1 -> UnitConverter804/1
  UnitConverter804/1 -> VOUTP_EC1EMSupTSC1CtrlPG1_cnt/1  "VOUTP_EC1EMSupTSC1CtrlPG1_cnt"
  VTQD_EC1EMSupTSC1CtrlPG3_cnt/1 -> VTQD_EC1EMSupTSC1CtrlPG3_cnt_Inproc/1  "VTQD_EC1EMSupTSC1CtrlPG3_cnt"
  VTQD_EC1EMSupTSC1CtrlPG3_cnt_Inproc/1 -> UnitConverter805/1
  UnitConverter805/1 -> VOUTP_EC1EMSupTSC1CtrlPG3_cnt/1  "VOUTP_EC1EMSupTSC1CtrlPG3_cnt"
  VTQD_EC1EMSupTSC1CtrlPG2_cnt/1 -> VTQD_EC1EMSupTSC1CtrlPG2_cnt_Inproc/1  "VTQD_EC1EMSupTSC1CtrlPG2_cnt"
  VTQD_EC1EMSupTSC1CtrlPG2_cnt_Inproc/1 -> UnitConverter806/1
  UnitConverter806/1 -> VOUTP_EC1EMSupTSC1CtrlPG2_cnt/1  "VOUTP_EC1EMSupTSC1CtrlPG2_cnt"
  VTQD_EC1EMSupTSC1CtrlPG4_cnt/1 -> VTQD_EC1EMSupTSC1CtrlPG4_cnt_Inproc/1  "VTQD_EC1EMSupTSC1CtrlPG4_cnt"
  VTQD_EC1EMSupTSC1CtrlPG4_cnt_Inproc/1 -> UnitConverter807/1
  UnitConverter807/1 -> VOUTP_EC1EMSupTSC1CtrlPG4_cnt/1  "VOUTP_EC1EMSupTSC1CtrlPG4_cnt"
  VTQD_EC1EMSpdHdleP6_rpm/1 -> VTQD_EC1EMSpdHdleP6_rpm_Inproc/1  "VTQD_EC1EMSpdHdleP6_rpm"
  VTQD_EC1EMSpdHdleP6_rpm_Inproc/1 -> UnitConverter808/1
  UnitConverter808/1 -> VOUTP_EC1EMSpdHdleP6_rpm/1  "VOUTP_EC1EMSpdHdleP6_rpm"
  VTQD_EC1EMGainEndSpdGvn_gain/1 -> VTQD_EC1EMGainEndSpdGvn_gain_Inproc/1  "VTQD_EC1EMGainEndSpdGvn_gain"
  VTQD_EC1EMGainEndSpdGvn_gain_Inproc/1 -> UnitConverter809/1
  UnitConverter809/1 -> VOUTP_EC1EMGainEndSpdGvn_gain/1  "VOUTP_EC1EMGainEndSpdGvn_gain"
  VTQD_RC1RetType_enum/1 -> VTQD_RC1RetType_enum_Inproc/1  "VTQD_RC1RetType_enum"
  VTQD_RC1RetType_enum_Inproc/1 -> UnitConverter810/1
  UnitConverter810/1 -> VOUTP_RC1RetType_enum/1  "VOUTP_RC1RetType_enum"
  VTQD_RC1RetLocat_enum/1 -> VTQD_RC1RetLocat_enum_Inproc/1  "VTQD_RC1RetLocat_enum"
  VTQD_RC1RetLocat_enum_Inproc/1 -> UnitConverter811/1
  UnitConverter811/1 -> VOUTP_RC1RetLocat_enum/1  "VOUTP_RC1RetLocat_enum"
  VTQD_RC1RetCtrlMth_enum/1 -> VTQD_RC1RetCtrlMth_enum_Inproc/1  "VTQD_RC1RetCtrlMth_enum"
  VTQD_RC1RetCtrlMth_enum_Inproc/1 -> UnitConverter812/1
  UnitConverter812/1 -> VOUTP_RC1RetCtrlMth_enum/1  "VOUTP_RC1RetCtrlMth_enum"
  VTQD_RC1RetSpdIdleP1_rpm/1 -> VTQD_RC1RetSpdIdleP1_rpm_Inproc/1  "VTQD_RC1RetSpdIdleP1_rpm"
  VTQD_RC1RetSpdIdleP1_rpm_Inproc/1 -> UnitConverter813/1
  UnitConverter813/1 -> VOUTP_RC1RetSpdIdleP1_rpm/1  "VOUTP_RC1RetSpdIdleP1_rpm"
  VTQD_RC1PctTrqIdleP1_pct/1 -> VTQD_RC1PctTrqIdleP1_pct_Inproc/1  "VTQD_RC1PctTrqIdleP1_pct"
  VTQD_RC1PctTrqIdleP1_pct_Inproc/1 -> UnitConverter814/1
  UnitConverter814/1 -> VOUTP_RC1PctTrqIdleP1_pct/1  "VOUTP_RC1PctTrqIdleP1_pct"
  VTQD_RC1MaxRetSpdP2_rpm/1 -> VTQD_RC1MaxRetSpdP2_rpm_Inproc/1  "VTQD_RC1MaxRetSpdP2_rpm"
  VTQD_RC1MaxRetSpdP2_rpm_Inproc/1 -> UnitConverter815/1
  UnitConverter815/1 -> VOUTP_RC1MaxRetSpdP2_rpm/1  "VOUTP_RC1MaxRetSpdP2_rpm"
  VTQD_RC1RetSpdP2_pct/1 -> VTQD_RC1RetSpdP2_pct_Inproc/1  "VTQD_RC1RetSpdP2_pct"
  VTQD_RC1RetSpdP2_pct_Inproc/1 -> UnitConverter816/1
  UnitConverter816/1 -> VOUTP_RC1RetSpdP2_pct/1  "VOUTP_RC1RetSpdP2_pct"
  VTQD_RC1MaxRetSpdP3_rpm/1 -> VTQD_RC1MaxRetSpdP3_rpm_Inproc/1  "VTQD_RC1MaxRetSpdP3_rpm"
  VTQD_RC1MaxRetSpdP3_rpm_Inproc/1 -> UnitConverter817/1
  UnitConverter817/1 -> VOUTP_RC1MaxRetSpdP3_rpm/1  "VOUTP_RC1MaxRetSpdP3_rpm"
  VTQD_RC1PctTrqP3_pct/1 -> VTQD_RC1PctTrqP3_pct_Inproc/1  "VTQD_RC1PctTrqP3_pct"
  VTQD_RC1PctTrqP3_pct_Inproc/1 -> UnitConverter818/1
  UnitConverter818/1 -> VOUTP_RC1PctTrqP3_pct/1  "VOUTP_RC1PctTrqP3_pct"
  VTQD_RC1RefRetTrq_Nm/1 -> VTQD_RC1RefRetTrq_Nm_Inproc/1  "VTQD_RC1RefRetTrq_Nm"
  VTQD_RC1RefRetTrq_Nm_Inproc/1 -> UnitConverter819/1
  UnitConverter819/1 -> VOUTP_RC1RefRetTrq_Nm/1  "VOUTP_RC1RefRetTrq_Nm"
  VTQD_RC1RetSpdPekTrqP5_Nm/1 -> VTQD_RC1RetSpdPekTrqP5_Nm_Inproc/1  "VTQD_RC1RetSpdPekTrqP5_Nm"
  VTQD_RC1RetSpdPekTrqP5_Nm_Inproc/1 -> UnitConverter820/1
  UnitConverter820/1 -> VOUTP_RC1RetSpdPekTrqP5_Nm/1  "VOUTP_RC1RetSpdPekTrqP5_Nm"
  VTQD_RC1RetSpdP4_rpm/1 -> VTQD_RC1RetSpdP4_rpm_Inproc/1  "VTQD_RC1RetSpdP4_rpm"
  VTQD_RC1RetSpdP4_rpm_Inproc/1 -> UnitConverter821/1
  UnitConverter821/1 -> VOUTP_RC1RetSpdP4_rpm/1  "VOUTP_RC1RetSpdP4_rpm"
  VTQD_VCUMCUDemLoNegVal_rpm/1 -> VTQD_VCUMCUDemLoNegVal_rpm_Inproc/1  "VTQD_VCUMCUDemLoNegVal_rpm"
  VTQD_VCUMCUDemLoNegVal_rpm_Inproc/1 -> UnitConverter822/1
  UnitConverter822/1 -> VOUTP_VCUMCUDemLoNegVal_rpm/1  "VOUTP_VCUMCUDemLoNegVal_rpm"
  VTQD_VCUMCUDemSpd_rpm/1 -> VTQD_VCUMCUDemSpd_rpm_Inproc/1  "VTQD_VCUMCUDemSpd_rpm"
  VTQD_VCUMCUDemSpd_rpm_Inproc/1 -> UnitConverter823/1
  UnitConverter823/1 -> VOUTP_VCUMCUDemSpd_rpm/1  "VOUTP_VCUMCUDemSpd_rpm"
  VTQD_VCUMCUGearSta_enum/1 -> VTQD_VCUMCUGearSta_enum_Inproc/1  "VTQD_VCUMCUGearSta_enum"
  VTQD_VCUMCUGearSta_enum_Inproc/1 -> UnitConverter824/1
  UnitConverter824/1 -> VOUTP_VCUMCUGearSta_enum/1  "VOUTP_VCUMCUGearSta_enum"
  VTQD_TUpAIND_enum/1 -> VTQD_TUpAIND_enum_Inproc/1  "VTQD_TUpAIND_enum"
  VTQD_TUpAIND_enum_Inproc/1 -> UnitConverter825/1
  UnitConverter825/1 -> VOUTP_TUpAIND_enum/1  "VOUTP_TUpAIND_enum"
  VTQD_ETC1ShiftrPgs_enum/1 -> VTQD_ETC1ShiftrPgs_enum_Inproc/1  "VTQD_ETC1ShiftrPgs_enum"
  VTQD_ETC1ShiftrPgs_enum_Inproc/1 -> UnitConverter826/1
  UnitConverter826/1 -> VOUTP_ETC1ShiftrPgs_enum/1  "VOUTP_ETC1ShiftrPgs_enum"
  VTQD_EVCU1RecuperHighSta_enum/1 -> VTQD_EVCU1RecuperHighSta_enum_Inproc/1  "VTQD_EVCU1RecuperHighSta_enum"
  VTQD_EVCU1RecuperHighSta_enum_Inproc/1 -> UnitConverter827/1
  UnitConverter827/1 -> VOUTP_EVCU1RecuperHighSta_enum/1  "VOUTP_EVCU1RecuperHighSta_enum"
  VTQD_EMRC1DrvDemEMRtapTrq_pct/1 -> VTQD_EMRC1DrvDemEMRtapTrq_pct_Inproc/1  "VTQD_EMRC1DrvDemEMRtapTrq_pct"
  VTQD_EMRC1DrvDemEMRtapTrq_pct_Inproc/1 -> UnitConverter828/1
  UnitConverter828/1 -> VOUTP_EMRC1DrvDemEMRtapTrq_pct/1  "VOUTP_EMRC1DrvDemEMRtapTrq_pct"
  VTQD_EMRC1RetSelNonEng_pct/1 -> VTQD_EMRC1RetSelNonEng_pct_Inproc/1  "VTQD_EMRC1RetSelNonEng_pct"
  VTQD_EMRC1RetSelNonEng_pct_Inproc/1 -> UnitConverter829/1
  UnitConverter829/1 -> VOUTP_EMRC1RetSelNonEng_pct/1  "VOUTP_EMRC1RetSelNonEng_pct"
  VTQD_EMRC1SACtrlDev_cnt/1 -> VTQD_EMRC1SACtrlDev_cnt_Inproc/1  "VTQD_EMRC1SACtrlDev_cnt"
  VTQD_EMRC1SACtrlDev_cnt_Inproc/1 -> UnitConverter830/1
  UnitConverter830/1 -> VOUTP_EMRC1SACtrlDev_cnt/1  "VOUTP_EMRC1SACtrlDev_cnt"
  VTQD_VCUMCUHandBrk_flg/1 -> VTQD_VCUMCUHandBrk_flg_Inproc/1  "VTQD_VCUMCUHandBrk_flg"
  VTQD_VCUMCUHandBrk_flg_Inproc/1 -> UnitConverter831/1
  UnitConverter831/1 -> VOUTP_VCUMCUHandBrk_flg/1  "VOUTP_VCUMCUHandBrk_flg"
  VTQD_VCUMCUFootBrk_flg/1 -> VTQD_VCUMCUFootBrk_flg_Inproc/1  "VTQD_VCUMCUFootBrk_flg"
  VTQD_VCUMCUFootBrk_flg_Inproc/1 -> UnitConverter832/1
  UnitConverter832/1 -> VOUTP_VCUMCUFootBrk_flg/1  "VOUTP_VCUMCUFootBrk_flg"
  VTQR_FrTMTqReq_Nm/1 -> VTQR_FrTMTqReq_Nm_Inproc/1  "VTQR_FrTMTqReq_Nm"
  VTQR_FrTMTqReq_Nm_Inproc/1 -> UnitConverter833/1
  UnitConverter833/1 -> VOUTP_FrTMTqReq_Nm/1  "VOUTP_FrTMTqReq_Nm"
  VTQR_RrTMTqReq_Nm/1 -> VTQR_RrTMTqReq_Nm_Inproc/1  "VTQR_RrTMTqReq_Nm"
  VTQR_RrTMTqReq_Nm_Inproc/1 -> UnitConverter834/1
  UnitConverter834/1 -> VOUTP_RrTMTqReq_Nm/1  "VOUTP_RrTMTqReq_Nm"
  VV2L_ReqOBCV2LEna_enum/1 -> VV2L_ReqOBCV2LEna_enum_Inproc/1  "VV2L_ReqOBCV2LEna_enum"
  VV2L_ReqOBCV2LEna_enum_Inproc/1 -> UnitConverter835/1
  UnitConverter835/1 -> VOUTP_ReqOBCV2LEna_enum/1  "VOUTP_ReqOBCV2LEna_enum"
  VV2L_ReqV2LIVIPopup_enum/1 -> VV2L_ReqV2LIVIPopup_enum_Inproc/1  "VV2L_ReqV2LIVIPopup_enum"
  VV2L_ReqV2LIVIPopup_enum_Inproc/1 -> UnitConverter836/1
  UnitConverter836/1 -> VOUTP_ReqV2LIVIPopup_enum/1  "VOUTP_ReqV2LIVIPopup_enum"
  VV2L_ReqV2LIVIDisChrg_enum/1 -> VV2L_ReqV2LIVIDisChrg_enum_Inproc/1  "VV2L_ReqV2LIVIDisChrg_enum"
  VV2L_ReqV2LIVIDisChrg_enum_Inproc/1 -> UnitConverter837/1
  UnitConverter837/1 -> VOUTP_ReqV2LIVIDisChrg_enum/1  "VOUTP_ReqV2LIVIDisChrg_enum"
  VV2L_ReqOBCExtrV2LEna_enum/1 -> VV2L_ReqOBCExtrV2LEna_enum_Inproc/1  "VV2L_ReqOBCExtrV2LEna_enum"
  VV2L_ReqOBCExtrV2LEna_enum_Inproc/1 -> UnitConverter838/1
  UnitConverter838/1 -> VOUTP_ReqOBCExtrV2LEna_enum/1  "VOUTP_ReqOBCExtrV2LEna_enum"
  VV2L_ReqOBCIntrV2LEna_enum/1 -> VV2L_ReqOBCIntrV2LEna_enum_Inproc/1  "VV2L_ReqOBCIntrV2LEna_enum"
  VV2L_ReqOBCIntrV2LEna_enum_Inproc/1 -> UnitConverter839/1
  UnitConverter839/1 -> VOUTP_ReqOBCIntrV2LEna_enum/1  "VOUTP_ReqOBCIntrV2LEna_enum"
  VV2L_HVPO120VGrpALDSt_enum/1 -> VV2L_HVPO120VGrpALDSt_enum_Inproc/1  "VV2L_HVPO120VGrpALDSt_enum"
  VV2L_HVPO120VGrpALDSt_enum_Inproc/1 -> UnitConverter840/1
  UnitConverter840/1 -> VOUTP_HVPO120VGrpALDSt_enum/1  "VOUTP_HVPO120VGrpALDSt_enum"
  VV2L_HVPO120VGrpBLDSt_enum/1 -> VV2L_HVPO120VGrpBLDSt_enum_Inproc/1  "VV2L_HVPO120VGrpBLDSt_enum"
  VV2L_HVPO120VGrpBLDSt_enum_Inproc/1 -> UnitConverter841/1
  UnitConverter841/1 -> VOUTP_HVPO120VGrpBLDSt_enum/1  "VOUTP_HVPO120VGrpBLDSt_enum"
  VVMC_FeatSetSpdFinal_raw32/1 -> VVMC_FeatSetSpdFinal_raw32_Inproc/1  "VVMC_FeatSetSpdFinal_raw32"
  VVMC_FeatSetSpdFinal_raw32_Inproc/1 -> UnitConverter842/1
  UnitConverter842/1 -> VOUTP_FeatSetSpdFinal_raw32/1  "VOUTP_FeatSetSpdFinal_raw32"
  VVMC_VehicleSpeed_mph/1 -> VVMC_VehicleSpeed_mph_Inproc/1  "VVMC_VehicleSpeed_mph"
  VVMC_VehicleSpeed_mph_Inproc/1 -> UnitConverter843/1
  UnitConverter843/1 -> VOUTP_VehicleSpeed_mph/1  "VOUTP_VehicleSpeed_mph"
  VVMC_VehicleSpeed_kph/1 -> VVMC_VehicleSpeed_kph_Inproc/1  "VVMC_VehicleSpeed_kph"
  VVMC_VehicleSpeed_kph_Inproc/1 -> UnitConverter844/1
  UnitConverter844/1 -> VOUTP_VehicleSpeed_kph/1  "VOUTP_VehicleSpeed_kph"
  VVMC_MeterIndSpeed_raw32/1 -> VVMC_MeterIndSpeed_raw32_Inproc/1  "VVMC_MeterIndSpeed_raw32"
  VVMC_MeterIndSpeed_raw32_Inproc/1 -> UnitConverter845/1
  UnitConverter845/1 -> VOUTP_MeterIndSpeed_raw32/1  "VOUTP_MeterIndSpeed_raw32"
  VVMC_VMCAEBCtrlAvail_flg/1 -> VVMC_VMCAEBCtrlAvail_flg_Inproc/1  "VVMC_VMCAEBCtrlAvail_flg"
  VVMC_VMCAEBCtrlAvail_flg_Inproc/1 -> UnitConverter846/1
  UnitConverter846/1 -> VOUTP_VMCAEBCtrlAvail_flg/1  "VOUTP_VMCAEBCtrlAvail_flg"
  VVMC_VMCACCCtrlAvail_flg/1 -> VVMC_VMCACCCtrlAvail_flg_Inproc/1  "VVMC_VMCACCCtrlAvail_flg"
  VVMC_VMCACCCtrlAvail_flg_Inproc/1 -> UnitConverter847/1
  UnitConverter847/1 -> VOUTP_VMCACCCtrlAvail_flg/1  "VOUTP_VMCACCCtrlAvail_flg"
  VVMC_VMCCCCtrlAvail_flg/1 -> VVMC_VMCCCCtrlAvail_flg_Inproc/1  "VVMC_VMCCCCtrlAvail_flg"
  VVMC_VMCCCCtrlAvail_flg_Inproc/1 -> UnitConverter848/1
  UnitConverter848/1 -> VOUTP_VMCCCCtrlAvail_flg/1  "VOUTP_VMCCCCtrlAvail_flg"
  VVMC_VMCMSACtrlAvail_flg/1 -> VVMC_VMCMSACtrlAvail_flg_Inproc/1  "VVMC_VMCMSACtrlAvail_flg"
  VVMC_VMCMSACtrlAvail_flg_Inproc/1 -> UnitConverter849/1
  UnitConverter849/1 -> VOUTP_VMCMSACtrlAvail_flg/1  "VOUTP_VMCMSACtrlAvail_flg"
  VVMC_FeatArbitrSta_enum/1 -> VVMC_FeatArbitrSta_enum_Inproc/1  "VVMC_FeatArbitrSta_enum"
  VVMC_FeatArbitrSta_enum_Inproc/1 -> UnitConverter850/1
  UnitConverter850/1 -> VOUTP_FeatArbitrSta_enum/1  "VOUTP_FeatArbitrSta_enum"
  VVMC_FeatReqSpd_kph/1 -> VVMC_FeatReqSpd_kph_Inproc/1  "VVMC_FeatReqSpd_kph"
  VVMC_FeatReqSpd_kph_Inproc/1 -> UnitConverter851/1
  UnitConverter851/1 -> VOUTP_FeatReqSpd_kph/1  "VOUTP_FeatReqSpd_kph"
  VVMC_JerkPCT_pct/1 -> VVMC_JerkPCT_pct_Inproc/1  "VVMC_JerkPCT_pct"
  VVMC_JerkPCT_pct_Inproc/1 -> UnitConverter852/1
  UnitConverter852/1 -> VOUTP_JerkPCT_pct/1  "VOUTP_JerkPCT_pct"
  VVMC_LimitPCT_pct/1 -> VVMC_LimitPCT_pct_Inproc/1  "VVMC_LimitPCT_pct"
  VVMC_LimitPCT_pct_Inproc/1 -> UnitConverter853/1
  UnitConverter853/1 -> VOUTP_LimitPCT_pct/1  "VOUTP_LimitPCT_pct"
  VVMC_FrontRearSlipRatioCtrl_flg/1 -> VVMC_FrontRearSlipRatioCtrl_flg_Inproc/1  "VVMC_FrontRearSlipRatioCtrl_flg"
  VVMC_FrontRearSlipRatioCtrl_flg_Inproc/1 -> UnitConverter854/1
  UnitConverter854/1 -> VOUTP_FrontRearSlipRatioCtrl_flg/1  "VOUTP_FrontRearSlipRatioCtrl_flg"
  VVMC_RearWhlSlipRatioCtrl_flg/1 -> VVMC_RearWhlSlipRatioCtrl_flg_Inproc/1  "VVMC_RearWhlSlipRatioCtrl_flg"
  VVMC_RearWhlSlipRatioCtrl_flg_Inproc/1 -> UnitConverter855/1
  UnitConverter855/1 -> VOUTP_RearWhlSlipRatioCtrl_flg/1  "VOUTP_RearWhlSlipRatioCtrl_flg"
  VVMC_SingleWhlSlipRatioCtrl_flg/1 -> VVMC_SingleWhlSlipRatioCtrl_flg_Inproc/1  "VVMC_SingleWhlSlipRatioCtrl_flg"
  VVMC_SingleWhlSlipRatioCtrl_flg_Inproc/1 -> UnitConverter856/1
  UnitConverter856/1 -> VOUTP_SingleWhlSlipRatioCtrl_flg/1  "VOUTP_SingleWhlSlipRatioCtrl_flg"
  VVMC_LatAccCtrl_flg/1 -> VVMC_LatAccCtrl_flg_Inproc/1  "VVMC_LatAccCtrl_flg"
  VVMC_LatAccCtrl_flg_Inproc/1 -> UnitConverter857/1
  UnitConverter857/1 -> VOUTP_LatAccCtrl_flg/1  "VOUTP_LatAccCtrl_flg"
  VVMC_SafetyCtrl_flg/1 -> VVMC_SafetyCtrl_flg_Inproc/1  "VVMC_SafetyCtrl_flg"
  VVMC_SafetyCtrl_flg_Inproc/1 -> UnitConverter858/1
  UnitConverter858/1 -> VOUTP_SafetyCtrl_flg/1  "VOUTP_SafetyCtrl_flg"
  VVMC_SPD2ACCAct_flg/1 -> VVMC_SPD2ACCAct_flg_Inproc/1  "VVMC_SPD2ACCAct_flg"
  VVMC_SPD2ACCAct_flg_Inproc/1 -> UnitConverter859/1
  UnitConverter859/1 -> VOUTP_SPD2ACCAct_flg/1  "VOUTP_SPD2ACCAct_flg"
  VVMC_AccCalcuPID_mps2/1 -> VVMC_AccCalcuPID_mps2_Inproc/1  "VVMC_AccCalcuPID_mps2"
  VVMC_AccCalcuPID_mps2_Inproc/1 -> UnitConverter860/1
  UnitConverter860/1 -> VOUTP_AccCalcuPID_mps2/1  "VOUTP_AccCalcuPID_mps2"
  VVMC_ISOAccLimit_mps2/1 -> VVMC_ISOAccLimit_mps2_Inproc/1  "VVMC_ISOAccLimit_mps2"
  VVMC_ISOAccLimit_mps2_Inproc/1 -> UnitConverter861/1
  UnitConverter861/1 -> VOUTP_ISOAccLimit_mps2/1  "VOUTP_ISOAccLimit_mps2"
  VVMC_ISODecLimit_mps2/1 -> VVMC_ISODecLimit_mps2_Inproc/1  "VVMC_ISODecLimit_mps2"
  VVMC_ISODecLimit_mps2_Inproc/1 -> UnitConverter862/1
  UnitConverter862/1 -> VOUTP_ISODecLimit_mps2/1  "VOUTP_ISODecLimit_mps2"
  VVMC_ISOJerkLimit_mps3/1 -> VVMC_ISOJerkLimit_mps3_Inproc/1  "VVMC_ISOJerkLimit_mps3"
  VVMC_ISOJerkLimit_mps3_Inproc/1 -> UnitConverter863/1
  UnitConverter863/1 -> VOUTP_ISOJerkLimit_mps3/1  "VOUTP_ISOJerkLimit_mps3"
  VVMC_ACCRequiredAccel_mps2/1 -> VVMC_ACCRequiredAccel_mps2_Inproc/1  "VVMC_ACCRequiredAccel_mps2"
  VVMC_ACCRequiredAccel_mps2_Inproc/1 -> UnitConverter864/1
  UnitConverter864/1 -> VOUTP_ACCRequiredAccel_mps2/1  "VOUTP_ACCRequiredAccel_mps2"
  VVMC_DISCReqAcc_mps2/1 -> VVMC_DISCReqAcc_mps2_Inproc/1  "VVMC_DISCReqAcc_mps2"
  VVMC_DISCReqAcc_mps2_Inproc/1 -> UnitConverter865/1
  UnitConverter865/1 -> VOUTP_DISCReqAcc_mps2/1  "VOUTP_DISCReqAcc_mps2"
  VVMC_FeatArbitrFinal_enum/1 -> VVMC_FeatArbitrFinal_enum_Inproc/1  "VVMC_FeatArbitrFinal_enum"
  VVMC_FeatArbitrFinal_enum_Inproc/1 -> UnitConverter866/1
  UnitConverter866/1 -> VOUTP_FeatArbitrFinal_enum/1  "VOUTP_FeatArbitrFinal_enum"
  VVMC_ActACCRequiredAccel_mps2/1 -> VVMC_ActACCRequiredAccel_mps2_Inproc/1  "VVMC_ActACCRequiredAccel_mps2"
  VVMC_ActACCRequiredAccel_mps2_Inproc/1 -> UnitConverter867/1
  UnitConverter867/1 -> VOUTP_ActACCRequiredAccel_mps2/1  "VOUTP_ActACCRequiredAccel_mps2"
  VVMC_LateralCtrl_flg/1 -> VVMC_LateralCtrl_flg_Inproc/1  "VVMC_LateralCtrl_flg"
  VVMC_LateralCtrl_flg_Inproc/1 -> UnitConverter868/1
  UnitConverter868/1 -> VOUTP_LateralCtrl_flg/1  "VOUTP_LateralCtrl_flg"
  VVMC_ADASLKASta_enum/1 -> VVMC_ADASLKASta_enum_Inproc/1  "VVMC_ADASLKASta_enum"
  VVMC_ADASLKASta_enum_Inproc/1 -> UnitConverter869/1
  UnitConverter869/1 -> VOUTP_ADASLKASta_enum/1  "VOUTP_ADASLKASta_enum"
  VVMC_LKAStrToqReq_Nm/1 -> VVMC_LKAStrToqReq_Nm_Inproc/1  "VVMC_LKAStrToqReq_Nm"
  VVMC_LKAStrToqReq_Nm_Inproc/1 -> UnitConverter870/1
  UnitConverter870/1 -> VOUTP_LKAStrToqReq_Nm/1  "VOUTP_LKAStrToqReq_Nm"
  VVMC_LKATOIFault_flg/1 -> VVMC_LKATOIFault_flg_Inproc/1  "VVMC_LKATOIFault_flg"
  VVMC_LKATOIFault_flg_Inproc/1 -> UnitConverter871/1
  UnitConverter871/1 -> VOUTP_LKATOIFault_flg/1  "VOUTP_LKATOIFault_flg"
  VVMC_LKATOIAct_enum/1 -> VVMC_LKATOIAct_enum_Inproc/1  "VVMC_LKATOIAct_enum"
  VVMC_LKATOIAct_enum_Inproc/1 -> UnitConverter872/1
  UnitConverter872/1 -> VOUTP_LKATOIAct_enum/1  "VOUTP_LKATOIAct_enum"
  VVMC_ADASAEBReq_enum/1 -> VVMC_ADASAEBReq_enum_Inproc/1  "VVMC_ADASAEBReq_enum"
  VVMC_ADASAEBReq_enum_Inproc/1 -> UnitConverter873/1
  UnitConverter873/1 -> VOUTP_ADASAEBReq_enum/1  "VOUTP_ADASAEBReq_enum"
  VVMC_ADASFaultSta_flg/1 -> VVMC_ADASFaultSta_flg_Inproc/1  "VVMC_ADASFaultSta_flg"
  VVMC_ADASFaultSta_flg_Inproc/1 -> UnitConverter874/1
  UnitConverter874/1 -> VOUTP_ADASFaultSta_flg/1  "VOUTP_ADASFaultSta_flg"
  VVMC_AEBVehHoldReq_flg/1 -> VVMC_AEBVehHoldReq_flg_Inproc/1  "VVMC_AEBVehHoldReq_flg"
  VVMC_AEBVehHoldReq_flg_Inproc/1 -> UnitConverter875/1
  UnitConverter875/1 -> VOUTP_AEBVehHoldReq_flg/1  "VOUTP_AEBVehHoldReq_flg"
  VVMC_ACCVehHoldReq_flg/1 -> VVMC_ACCVehHoldReq_flg_Inproc/1  "VVMC_ACCVehHoldReq_flg"
  VVMC_ACCVehHoldReq_flg_Inproc/1 -> UnitConverter876/1
  UnitConverter876/1 -> VOUTP_ACCVehHoldReq_flg/1  "VOUTP_ACCVehHoldReq_flg"
  VVMC_ADASDBSReq_enum/1 -> VVMC_ADASDBSReq_enum_Inproc/1  "VVMC_ADASDBSReq_enum"
  VVMC_ADASDBSReq_enum_Inproc/1 -> UnitConverter877/1
  UnitConverter877/1 -> VOUTP_ADASDBSReq_enum/1  "VOUTP_ADASDBSReq_enum"
  VVMC_ADASACCSta_enum/1 -> VVMC_ADASACCSta_enum_Inproc/1  "VVMC_ADASACCSta_enum"
  VVMC_ADASACCSta_enum_Inproc/1 -> UnitConverter878/1
  UnitConverter878/1 -> VOUTP_ADASACCSta_enum/1  "VOUTP_ADASACCSta_enum"
  VVMC_ACCObjDist_m/1 -> VVMC_ACCObjDist_m_Inproc/1  "VVMC_ACCObjDist_m"
  VVMC_ACCObjDist_m_Inproc/1 -> UnitConverter879/1
  UnitConverter879/1 -> VOUTP_ACCObjDist_m/1  "VOUTP_ACCObjDist_m"
  VVMC_ACCObjRelSpd_mps/1 -> VVMC_ACCObjRelSpd_mps_Inproc/1  "VVMC_ACCObjRelSpd_mps"
  VVMC_ACCObjRelSpd_mps_Inproc/1 -> UnitConverter880/1
  UnitConverter880/1 -> VOUTP_ACCObjRelSpd_mps/1  "VOUTP_ACCObjRelSpd_mps"
  VVMC_TimeGapLevel_enum/1 -> VVMC_TimeGapLevel_enum_Inproc/1  "VVMC_TimeGapLevel_enum"
  VVMC_TimeGapLevel_enum_Inproc/1 -> UnitConverter881/1
  UnitConverter881/1 -> VOUTP_TimeGapLevel_enum/1  "VOUTP_TimeGapLevel_enum"
  VVMC_ACCJerkUpperLimit_mps3/1 -> VVMC_ACCJerkUpperLimit_mps3_Inproc/1  "VVMC_ACCJerkUpperLimit_mps3"
  VVMC_ACCJerkUpperLimit_mps3_Inproc/1 -> UnitConverter882/1
  UnitConverter882/1 -> VOUTP_ACCJerkUpperLimit_mps3/1  "VOUTP_ACCJerkUpperLimit_mps3"
  VVMC_ACCComfortBandUpper_mps2/1 -> VVMC_ACCComfortBandUpper_mps2_Inproc/1  "VVMC_ACCComfortBandUpper_mps2"
  VVMC_ACCComfortBandUpper_mps2_Inproc/1 -> UnitConverter883/1
  UnitConverter883/1 -> VOUTP_ACCComfortBandUpper_mps2/1  "VOUTP_ACCComfortBandUpper_mps2"
  VVMC_ACCJerkLowerLimit_mps3/1 -> VVMC_ACCJerkLowerLimit_mps3_Inproc/1  "VVMC_ACCJerkLowerLimit_mps3"
  VVMC_ACCJerkLowerLimit_mps3_Inproc/1 -> UnitConverter884/1
  UnitConverter884/1 -> VOUTP_ACCJerkLowerLimit_mps3/1  "VOUTP_ACCJerkLowerLimit_mps3"
  VVMC_ACCComfortBandLower_mps2/1 -> VVMC_ACCComfortBandLower_mps2_Inproc/1  "VVMC_ACCComfortBandLower_mps2"
  VVMC_ACCComfortBandLower_mps2_Inproc/1 -> UnitConverter885/1
  UnitConverter885/1 -> VOUTP_ACCComfortBandLower_mps2/1  "VOUTP_ACCComfortBandLower_mps2"
  VVMC_ADASVehSpdLim_raw32/1 -> VVMC_ADASVehSpdLim_raw32_Inproc/1  "VVMC_ADASVehSpdLim_raw32"
  VVMC_ADASVehSpdLim_raw32_Inproc/1 -> UnitConverter886/1
  UnitConverter886/1 -> VOUTP_ADASVehSpdLim_raw32/1  "VOUTP_ADASVehSpdLim_raw32"
  VVMC_ADASShftPosnReqA_flg/1 -> VVMC_ADASShftPosnReqA_flg_Inproc/1  "VVMC_ADASShftPosnReqA_flg"
  VVMC_ADASShftPosnReqA_flg_Inproc/1 -> UnitConverter887/1
  UnitConverter887/1 -> VOUTP_ADASShftPosnReqA_flg/1  "VOUTP_ADASShftPosnReqA_flg"
  VVMC_ADASShftPosnReq_enum/1 -> VVMC_ADASShftPosnReq_enum_Inproc/1  "VVMC_ADASShftPosnReq_enum"
  VVMC_ADASShftPosnReq_enum_Inproc/1 -> UnitConverter888/1
  UnitConverter888/1 -> VOUTP_ADASShftPosnReq_enum/1  "VOUTP_ADASShftPosnReq_enum"
  VVMC_ADASForceIdle_flg/1 -> VVMC_ADASForceIdle_flg_Inproc/1  "VVMC_ADASForceIdle_flg"
  VVMC_ADASForceIdle_flg_Inproc/1 -> UnitConverter889/1
  UnitConverter889/1 -> VOUTP_ADASForceIdle_flg/1  "VOUTP_ADASForceIdle_flg"
  VVMC_HazardWarningReq_flg/1 -> VVMC_HazardWarningReq_flg_Inproc/1  "VVMC_HazardWarningReq_flg"
  VVMC_HazardWarningReq_flg_Inproc/1 -> UnitConverter890/1
  UnitConverter890/1 -> VOUTP_HazardWarningReq_flg/1  "VOUTP_HazardWarningReq_flg"
  VVMC_RightTurnLightReq_flg/1 -> VVMC_RightTurnLightReq_flg_Inproc/1  "VVMC_RightTurnLightReq_flg"
  VVMC_RightTurnLightReq_flg_Inproc/1 -> UnitConverter891/1
  UnitConverter891/1 -> VOUTP_RightTurnLightReq_flg/1  "VOUTP_RightTurnLightReq_flg"
  VVMC_LeftTurnLightReq_flg/1 -> VVMC_LeftTurnLightReq_flg_Inproc/1  "VVMC_LeftTurnLightReq_flg"
  VVMC_LeftTurnLightReq_flg_Inproc/1 -> UnitConverter892/1
  UnitConverter892/1 -> VOUTP_LeftTurnLightReq_flg/1  "VOUTP_LeftTurnLightReq_flg"
  VVMC_ADASFCWSta_enum/1 -> VVMC_ADASFCWSta_enum_Inproc/1  "VVMC_ADASFCWSta_enum"
  VVMC_ADASFCWSta_enum_Inproc/1 -> UnitConverter893/1
  UnitConverter893/1 -> VOUTP_ADASFCWSta_enum/1  "VOUTP_ADASFCWSta_enum"
  VVMC_ADASLDWSta_enum/1 -> VVMC_ADASLDWSta_enum_Inproc/1  "VVMC_ADASLDWSta_enum"
  VVMC_ADASLDWSta_enum_Inproc/1 -> UnitConverter894/1
  UnitConverter894/1 -> VOUTP_ADASLDWSta_enum/1  "VOUTP_ADASLDWSta_enum"
  VVMC_ADASFltWrnReq_flg/1 -> VVMC_ADASFltWrnReq_flg_Inproc/1  "VVMC_ADASFltWrnReq_flg"
  VVMC_ADASFltWrnReq_flg_Inproc/1 -> UnitConverter895/1
  UnitConverter895/1 -> VOUTP_ADASFltWrnReq_flg/1  "VOUTP_ADASFltWrnReq_flg"
  VVMC_ACCObjDstLvl_enum/1 -> VVMC_ACCObjDstLvl_enum_Inproc/1  "VVMC_ACCObjDstLvl_enum"
  VVMC_ACCObjDstLvl_enum_Inproc/1 -> UnitConverter896/1
  UnitConverter896/1 -> VOUTP_ACCObjDstLvl_enum/1  "VOUTP_ACCObjDstLvl_enum"
  VVMC_ForceLowBeam_enum/1 -> VVMC_ForceLowBeam_enum_Inproc/1  "VVMC_ForceLowBeam_enum"
  VVMC_ForceLowBeam_enum_Inproc/1 -> UnitConverter897/1
  UnitConverter897/1 -> VOUTP_ForceLowBeam_enum/1  "VOUTP_ForceLowBeam_enum"
  VVMC_ACCTakeoverReq_flg/1 -> VVMC_ACCTakeoverReq_flg_Inproc/1  "VVMC_ACCTakeoverReq_flg"
  VVMC_ACCTakeoverReq_flg_Inproc/1 -> UnitConverter898/1
  UnitConverter898/1 -> VOUTP_ACCTakeoverReq_flg/1  "VOUTP_ACCTakeoverReq_flg"
  VVMC_ADASWarningMsg_enum/1 -> VVMC_ADASWarningMsg_enum_Inproc/1  "VVMC_ADASWarningMsg_enum"
  VVMC_ADASWarningMsg_enum_Inproc/1 -> UnitConverter899/1
  UnitConverter899/1 -> VOUTP_ADASWarningMsg_enum/1  "VOUTP_ADASWarningMsg_enum"
  VVMC_ADASCAMSpdLim_enum/1 -> VVMC_ADASCAMSpdLim_enum_Inproc/1  "VVMC_ADASCAMSpdLim_enum"
  VVMC_ADASCAMSpdLim_enum_Inproc/1 -> UnitConverter900/1
  UnitConverter900/1 -> VOUTP_ADASCAMSpdLim_enum/1  "VOUTP_ADASCAMSpdLim_enum"
  VVMC_TargetType_enum/1 -> VVMC_TargetType_enum_Inproc/1  "VVMC_TargetType_enum"
  VVMC_TargetType_enum_Inproc/1 -> UnitConverter901/1
  UnitConverter901/1 -> VOUTP_TargetType_enum/1  "VOUTP_TargetType_enum"
  VVMC_ADASSLIFSpdLim_enum/1 -> VVMC_ADASSLIFSpdLim_enum_Inproc/1  "VVMC_ADASSLIFSpdLim_enum"
  VVMC_ADASSLIFSpdLim_enum_Inproc/1 -> UnitConverter902/1
  UnitConverter902/1 -> VOUTP_ADASSLIFSpdLim_enum/1  "VOUTP_ADASSLIFSpdLim_enum"
  VVMC_LKAHODDisplayWarning_flg/1 -> VVMC_LKAHODDisplayWarning_flg_Inproc/1  "VVMC_LKAHODDisplayWarning_flg"
  VVMC_LKAHODDisplayWarning_flg_Inproc/1 -> UnitConverter903/1
  UnitConverter903/1 -> VOUTP_LKAHODDisplayWarning_flg/1  "VOUTP_LKAHODDisplayWarning_flg"
  VVMC_LKAHODSoundWarning_flg/1 -> VVMC_LKAHODSoundWarning_flg_Inproc/1  "VVMC_LKAHODSoundWarning_flg"
  VVMC_LKAHODSoundWarning_flg_Inproc/1 -> UnitConverter904/1
  UnitConverter904/1 -> VOUTP_LKAHODSoundWarning_flg/1  "VOUTP_LKAHODSoundWarning_flg"
  VVMC_ADASLFCSta_enum/1 -> VVMC_ADASLFCSta_enum_Inproc/1  "VVMC_ADASLFCSta_enum"
  VVMC_ADASLFCSta_enum_Inproc/1 -> UnitConverter905/1
  UnitConverter905/1 -> VOUTP_ADASLFCSta_enum/1  "VOUTP_ADASLFCSta_enum"
  VVMC_ADASLaneModeL_enum/1 -> VVMC_ADASLaneModeL_enum_Inproc/1  "VVMC_ADASLaneModeL_enum"
  VVMC_ADASLaneModeL_enum_Inproc/1 -> UnitConverter906/1
  UnitConverter906/1 -> VOUTP_ADASLaneModeL_enum/1  "VOUTP_ADASLaneModeL_enum"
  VVMC_ADASLaneModeR_enum/1 -> VVMC_ADASLaneModeR_enum_Inproc/1  "VVMC_ADASLaneModeR_enum"
  VVMC_ADASLaneModeR_enum_Inproc/1 -> UnitConverter907/1
  UnitConverter907/1 -> VOUTP_ADASLaneModeR_enum/1  "VOUTP_ADASLaneModeR_enum"
  VVMC_ADASSLIFSta_enum/1 -> VVMC_ADASSLIFSta_enum_Inproc/1  "VVMC_ADASSLIFSta_enum"
  VVMC_ADASSLIFSta_enum_Inproc/1 -> UnitConverter908/1
  UnitConverter908/1 -> VOUTP_ADASSLIFSta_enum/1  "VOUTP_ADASSLIFSta_enum"
  VVMC_ADASISASta_enum/1 -> VVMC_ADASISASta_enum_Inproc/1  "VVMC_ADASISASta_enum"
  VVMC_ADASISASta_enum_Inproc/1 -> UnitConverter909/1
  UnitConverter909/1 -> VOUTP_ADASISASta_enum/1  "VOUTP_ADASISASta_enum"
  VVMC_ADASLDWMute_flg/1 -> VVMC_ADASLDWMute_flg_Inproc/1  "VVMC_ADASLDWMute_flg"
  VVMC_ADASLDWMute_flg_Inproc/1 -> UnitConverter910/1
  UnitConverter910/1 -> VOUTP_ADASLDWMute_flg/1  "VOUTP_ADASLDWMute_flg"
  VVMC_ADASFCWMute_flg/1 -> VVMC_ADASFCWMute_flg_Inproc/1  "VVMC_ADASFCWMute_flg"
  VVMC_ADASFCWMute_flg_Inproc/1 -> UnitConverter911/1
  UnitConverter911/1 -> VOUTP_ADASFCWMute_flg/1  "VOUTP_ADASFCWMute_flg"
  VVMC_ADASLFCHandsOffWarning_enum/1 -> VVMC_ADASLFCHandsOffWarning_enum_Inproc/1  "VVMC_ADASLFCHandsOffWarning_enum"
  VVMC_ADASLFCHandsOffWarning_enum_Inproc/1 -> UnitConverter912/1
  UnitConverter912/1 -> VOUTP_ADASLFCHandsOffWarning_enum/1  "VOUTP_ADASLFCHandsOffWarning_enum"
  VVMC_LVDADisabled_flg/1 -> VVMC_LVDADisabled_flg_Inproc/1  "VVMC_LVDADisabled_flg"
  VVMC_LVDADisabled_flg_Inproc/1 -> UnitConverter913/1
  UnitConverter913/1 -> VOUTP_LVDADisabled_flg/1  "VOUTP_LVDADisabled_flg"
  VVMC_LVDAMuteSta_enum/1 -> VVMC_LVDAMuteSta_enum_Inproc/1  "VVMC_LVDAMuteSta_enum"
  VVMC_LVDAMuteSta_enum_Inproc/1 -> UnitConverter914/1
  UnitConverter914/1 -> VOUTP_LVDAMuteSta_enum/1  "VOUTP_LVDAMuteSta_enum"
  VVMC_LVDAFailinfo_flg/1 -> VVMC_LVDAFailinfo_flg_Inproc/1  "VVMC_LVDAFailinfo_flg"
  VVMC_LVDAFailinfo_flg_Inproc/1 -> UnitConverter915/1
  UnitConverter915/1 -> VOUTP_LVDAFailinfo_flg/1  "VOUTP_LVDAFailinfo_flg"
  VVMC_LVDAWarning_flg/1 -> VVMC_LVDAWarning_flg_Inproc/1  "VVMC_LVDAWarning_flg"
  VVMC_LVDAWarning_flg_Inproc/1 -> UnitConverter916/1
  UnitConverter916/1 -> VOUTP_LVDAWarning_flg/1  "VOUTP_LVDAWarning_flg"
  VVMC_LVDAACCStatusInformation_flg/1 -> VVMC_LVDAACCStatusInformation_flg_Inproc/1  "VVMC_LVDAACCStatusInformation_flg"
  VVMC_LVDAACCStatusInformation_flg_Inproc/1 -> UnitConverter917/1
  UnitConverter917/1 -> VOUTP_LVDAACCStatusInformation_flg/1  "VOUTP_LVDAACCStatusInformation_flg"
  VVMC_ADASLFCWarnSound_enum/1 -> VVMC_ADASLFCWarnSound_enum_Inproc/1  "VVMC_ADASLFCWarnSound_enum"
  VVMC_ADASLFCWarnSound_enum_Inproc/1 -> UnitConverter918/1
  UnitConverter918/1 -> VOUTP_ADASLFCWarnSound_enum/1  "VOUTP_ADASLFCWarnSound_enum"
  VVMC_FCMACCmode_enum/1 -> VVMC_FCMACCmode_enum_Inproc/1  "VVMC_FCMACCmode_enum"
  VVMC_FCMACCmode_enum_Inproc/1 -> UnitConverter919/1
  UnitConverter919/1 -> VOUTP_FCMACCmode_enum/1  "VOUTP_FCMACCmode_enum"
  VVMC_ADASLanetypeR_enum/1 -> VVMC_ADASLanetypeR_enum_Inproc/1  "VVMC_ADASLanetypeR_enum"
  VVMC_ADASLanetypeR_enum_Inproc/1 -> UnitConverter920/1
  UnitConverter920/1 -> VOUTP_ADASLanetypeR_enum/1  "VOUTP_ADASLanetypeR_enum"
  VVMC_ADASLanetypeL_enum/1 -> VVMC_ADASLanetypeL_enum_Inproc/1  "VVMC_ADASLanetypeL_enum"
  VVMC_ADASLanetypeL_enum_Inproc/1 -> UnitConverter921/1
  UnitConverter921/1 -> VOUTP_ADASLanetypeL_enum/1  "VOUTP_ADASLanetypeL_enum"
  VVMC_ADASLanecurveL_raw32/1 -> VVMC_ADASLanecurveL_raw32_Inproc/1  "VVMC_ADASLanecurveL_raw32"
  VVMC_ADASLanecurveL_raw32_Inproc/1 -> UnitConverter922/1
  UnitConverter922/1 -> VOUTP_ADASLanecurveL_raw32/1  "VOUTP_ADASLanecurveL_raw32"
  VVMC_ADASLanecurveR_raw32/1 -> VVMC_ADASLanecurveR_raw32_Inproc/1  "VVMC_ADASLanecurveR_raw32"
  VVMC_ADASLanecurveR_raw32_Inproc/1 -> UnitConverter923/1
  UnitConverter923/1 -> VOUTP_ADASLanecurveR_raw32/1  "VOUTP_ADASLanecurveR_raw32"
  VVMC_ADASAEBSta_enum/1 -> VVMC_ADASAEBSta_enum_Inproc/1  "VVMC_ADASAEBSta_enum"
  VVMC_ADASAEBSta_enum_Inproc/1 -> UnitConverter924/1
  UnitConverter924/1 -> VOUTP_ADASAEBSta_enum/1  "VOUTP_ADASAEBSta_enum"
  VVMC_FCMLDWRequest_enum/1 -> VVMC_FCMLDWRequest_enum_Inproc/1  "VVMC_FCMLDWRequest_enum"
  VVMC_FCMLDWRequest_enum_Inproc/1 -> UnitConverter925/1
  UnitConverter925/1 -> VOUTP_FCMLDWRequest_enum/1  "VOUTP_FCMLDWRequest_enum"
  VVMC_FCMLDWFault_flg/1 -> VVMC_FCMLDWFault_flg_Inproc/1  "VVMC_FCMLDWFault_flg"
  VVMC_FCMLDWFault_flg_Inproc/1 -> UnitConverter926/1
  UnitConverter926/1 -> VOUTP_FCMLDWFault_flg/1  "VOUTP_FCMLDWFault_flg"
  VVMC_ACCCtrlAvail_flg/1 -> VVMC_ACCCtrlAvail_flg_Inproc/1  "VVMC_ACCCtrlAvail_flg"
  VVMC_ACCCtrlAvail_flg_Inproc/1 -> UnitConverter927/1
  UnitConverter927/1 -> VOUTP_ACCCtrlAvail_flg/1  "VOUTP_ACCCtrlAvail_flg"
  VVMC_ACCPedalOvrd_flg/1 -> VVMC_ACCPedalOvrd_flg_Inproc/1  "VVMC_ACCPedalOvrd_flg"
  VVMC_ACCPedalOvrd_flg_Inproc/1 -> UnitConverter928/1
  UnitConverter928/1 -> VOUTP_ACCPedalOvrd_flg/1  "VOUTP_ACCPedalOvrd_flg"
  VVMC_TimeGapCalcu_s/1 -> VVMC_TimeGapCalcu_s_Inproc/1  "VVMC_TimeGapCalcu_s"
  VVMC_TimeGapCalcu_s_Inproc/1 -> UnitConverter929/1
  UnitConverter929/1 -> VOUTP_TimeGapCalcu_s/1  "VOUTP_TimeGapCalcu_s"
  VVMC_CCCtrlSta_enum/1 -> VVMC_CCCtrlSta_enum_Inproc/1  "VVMC_CCCtrlSta_enum"
  VVMC_CCCtrlSta_enum_Inproc/1 -> UnitConverter930/1
  UnitConverter930/1 -> VOUTP_CCCtrlSta_enum/1  "VOUTP_CCCtrlSta_enum"
  VVMC_MSACtrlSta_enum/1 -> VVMC_MSACtrlSta_enum_Inproc/1  "VVMC_MSACtrlSta_enum"
  VVMC_MSACtrlSta_enum_Inproc/1 -> UnitConverter931/1
  UnitConverter931/1 -> VOUTP_MSACtrlSta_enum/1  "VOUTP_MSACtrlSta_enum"
  VVMC_APSCtrlAvail_flg/1 -> VVMC_APSCtrlAvail_flg_Inproc/1  "VVMC_APSCtrlAvail_flg"
  VVMC_APSCtrlAvail_flg_Inproc/1 -> UnitConverter932/1
  UnitConverter932/1 -> VOUTP_APSCtrlAvail_flg/1  "VOUTP_APSCtrlAvail_flg"
  VVMC_APSActive_flg/1 -> VVMC_APSActive_flg_Inproc/1  "VVMC_APSActive_flg"
  VVMC_APSActive_flg_Inproc/1 -> UnitConverter933/1
  UnitConverter933/1 -> VOUTP_APSActive_flg/1  "VOUTP_APSActive_flg"
  VVMC_APSStaSys_enum/1 -> VVMC_APSStaSys_enum_Inproc/1  "VVMC_APSStaSys_enum"
  VVMC_APSStaSys_enum_Inproc/1 -> UnitConverter934/1
  UnitConverter934/1 -> VOUTP_APSStaSys_enum/1  "VOUTP_APSStaSys_enum"
  VVMC_APSDecReqA_flg/1 -> VVMC_APSDecReqA_flg_Inproc/1  "VVMC_APSDecReqA_flg"
  VVMC_APSDecReqA_flg_Inproc/1 -> UnitConverter935/1
  UnitConverter935/1 -> VOUTP_APSDecReqA_flg/1  "VOUTP_APSDecReqA_flg"
  VVMC_APSDecReq_mps2/1 -> VVMC_APSDecReq_mps2_Inproc/1  "VVMC_APSDecReq_mps2"
  VVMC_APSDecReq_mps2_Inproc/1 -> UnitConverter936/1
  UnitConverter936/1 -> VOUTP_APSDecReq_mps2/1  "VOUTP_APSDecReq_mps2"
  VVMC_APSReq_enum/1 -> VVMC_APSReq_enum_Inproc/1  "VVMC_APSReq_enum"
  VVMC_APSReq_enum_Inproc/1 -> UnitConverter937/1
  UnitConverter937/1 -> VOUTP_APSReq_enum/1  "VOUTP_APSReq_enum"
  VVMC_LongAcc_Gps/1 -> VVMC_LongAcc_Gps_Inproc/1  "VVMC_LongAcc_Gps"
  VVMC_LongAcc_Gps_Inproc/1 -> UnitConverter938/1
  UnitConverter938/1 -> VOUTP_LongAcc_Gps/1  "VOUTP_LongAcc_Gps"
  VVMC_CCMSASpdWar_flg/1 -> VVMC_CCMSASpdWar_flg_Inproc/1  "VVMC_CCMSASpdWar_flg"
  VVMC_CCMSASpdWar_flg_Inproc/1 -> UnitConverter939/1
  UnitConverter939/1 -> VOUTP_CCMSASpdWar_flg/1  "VOUTP_CCMSASpdWar_flg"
  VVMC_IMUEnaCmd_flg/1 -> VVMC_IMUEnaCmd_flg_Inproc/1  "VVMC_IMUEnaCmd_flg"
  VVMC_IMUEnaCmd_flg_Inproc/1 -> UnitConverter940/1
  UnitConverter940/1 -> VOUTP_IMUEnaCmd_flg/1  "VOUTP_IMUEnaCmd_flg"
  VVMC_CAASCtrlAvail_flg/1 -> VVMC_CAASCtrlAvail_flg_Inproc/1  "VVMC_CAASCtrlAvail_flg"
  VVMC_CAASCtrlAvail_flg_Inproc/1 -> UnitConverter941/1
  UnitConverter941/1 -> VOUTP_CAASCtrlAvail_flg/1  "VOUTP_CAASCtrlAvail_flg"
  VVMC_CAASActive_flg/1 -> VVMC_CAASActive_flg_Inproc/1  "VVMC_CAASActive_flg"
  VVMC_CAASActive_flg_Inproc/1 -> UnitConverter942/1
  UnitConverter942/1 -> VOUTP_CAASActive_flg/1  "VOUTP_CAASActive_flg"
  VVMC_ExtraMSACtrlSta_enum/1 -> VVMC_ExtraMSACtrlSta_enum_Inproc/1  "VVMC_ExtraMSACtrlSta_enum"
  VVMC_ExtraMSACtrlSta_enum_Inproc/1 -> UnitConverter943/1
  UnitConverter943/1 -> VOUTP_ExtraMSACtrlSta_enum/1  "VOUTP_ExtraMSACtrlSta_enum"
  VVMC_CalibratedAccX_G/1 -> VVMC_CalibratedAccX_G_Inproc/1  "VVMC_CalibratedAccX_G"
  VVMC_CalibratedAccX_G_Inproc/1 -> UnitConverter944/1
  UnitConverter944/1 -> VOUTP_CalibratedAccX_G/1  "VOUTP_CalibratedAccX_G"
  VVMC_CalibratedAccY_G/1 -> VVMC_CalibratedAccY_G_Inproc/1  "VVMC_CalibratedAccY_G"
  VVMC_CalibratedAccY_G_Inproc/1 -> UnitConverter945/1
  UnitConverter945/1 -> VOUTP_CalibratedAccY_G/1  "VOUTP_CalibratedAccY_G"
  VVMC_CalibratedAccZ_G/1 -> VVMC_CalibratedAccZ_G_Inproc/1  "VVMC_CalibratedAccZ_G"
  VVMC_CalibratedAccZ_G_Inproc/1 -> UnitConverter946/1
  UnitConverter946/1 -> VOUTP_CalibratedAccZ_G/1  "VOUTP_CalibratedAccZ_G"
  VVMC_CalibratedGyroX_Dps/1 -> VVMC_CalibratedGyroX_Dps_Inproc/1  "VVMC_CalibratedGyroX_Dps"
  VVMC_CalibratedGyroX_Dps_Inproc/1 -> UnitConverter947/1
  UnitConverter947/1 -> VOUTP_CalibratedGyroX_Dps/1  "VOUTP_CalibratedGyroX_Dps"
  VVMC_CalibratedGyroY_Dps/1 -> VVMC_CalibratedGyroY_Dps_Inproc/1  "VVMC_CalibratedGyroY_Dps"
  VVMC_CalibratedGyroY_Dps_Inproc/1 -> UnitConverter948/1
  UnitConverter948/1 -> VOUTP_CalibratedGyroY_Dps/1  "VOUTP_CalibratedGyroY_Dps"
  VVMC_CalibratedGyroZ_Dps/1 -> VVMC_CalibratedGyroZ_Dps_Inproc/1  "VVMC_CalibratedGyroZ_Dps"
  VVMC_CalibratedGyroZ_Dps_Inproc/1 -> UnitConverter949/1
  UnitConverter949/1 -> VOUTP_CalibratedGyroZ_Dps/1  "VOUTP_CalibratedGyroZ_Dps"
  VVMC_FDCVMCAPSVRqEPSCtrl_flg/1 -> VVMC_FDCVMCAPSVRqEPSCtrl_flg_Inproc/1  "VVMC_FDCVMCAPSVRqEPSCtrl_flg"
  VVMC_FDCVMCAPSVRqEPSCtrl_flg_Inproc/1 -> UnitConverter950/1
  UnitConverter950/1 -> VOUTP_FDCVMCAPSVRqEPSCtrl_flg/1  "VOUTP_FDCVMCAPSVRqEPSCtrl_flg"
  VVMC_FDCVMCAPSAngleTarget_deg/1 -> VVMC_FDCVMCAPSAngleTarget_deg_Inproc/1  "VVMC_FDCVMCAPSAngleTarget_deg"
  VVMC_FDCVMCAPSAngleTarget_deg_Inproc/1 -> UnitConverter951/1
  UnitConverter951/1 -> VOUTP_FDCVMCAPSAngleTarget_deg/1  "VOUTP_FDCVMCAPSAngleTarget_deg"
  VVMC_FDCVMCAPSRqEPSCtrl_flg/1 -> VVMC_FDCVMCAPSRqEPSCtrl_flg_Inproc/1  "VVMC_FDCVMCAPSRqEPSCtrl_flg"
  VVMC_FDCVMCAPSRqEPSCtrl_flg_Inproc/1 -> UnitConverter952/1
  UnitConverter952/1 -> VOUTP_FDCVMCAPSRqEPSCtrl_flg/1  "VOUTP_FDCVMCAPSRqEPSCtrl_flg"
  VVMC_FDCVMCAngCtrlTqWtGn_pct/1 -> VVMC_FDCVMCAngCtrlTqWtGn_pct_Inproc/1  "VVMC_FDCVMCAngCtrlTqWtGn_pct"
  VVMC_FDCVMCAngCtrlTqWtGn_pct_Inproc/1 -> UnitConverter953/1
  UnitConverter953/1 -> VOUTP_FDCVMCAngCtrlTqWtGn_pct/1  "VOUTP_FDCVMCAngCtrlTqWtGn_pct"
  VVMC_FDCVMCDrInpTqBstAct_flg/1 -> VVMC_FDCVMCDrInpTqBstAct_flg_Inproc/1  "VVMC_FDCVMCDrInpTqBstAct_flg"
  VVMC_FDCVMCDrInpTqBstAct_flg_Inproc/1 -> UnitConverter954/1
  UnitConverter954/1 -> VOUTP_FDCVMCDrInpTqBstAct_flg/1  "VOUTP_FDCVMCDrInpTqBstAct_flg"
  VVMC_FDCVMCMaxAngCtrlOutTqLim_Nm/1 -> VVMC_FDCVMCMaxAngCtrlOutTqLim_Nm_Inproc/1  "VVMC_FDCVMCMaxAngCtrlOutTqLim_Nm"
  VVMC_FDCVMCMaxAngCtrlOutTqLim_Nm_Inproc/1 -> UnitConverter955/1
  UnitConverter955/1 -> VOUTP_FDCVMCMaxAngCtrlOutTqLim_Nm/1  "VOUTP_FDCVMCMaxAngCtrlOutTqLim_Nm"
  VVMC_FDCVMCDrInpTqBstGn_pct/1 -> VVMC_FDCVMCDrInpTqBstGn_pct_Inproc/1  "VVMC_FDCVMCDrInpTqBstGn_pct"
  VVMC_FDCVMCDrInpTqBstGn_pct_Inproc/1 -> UnitConverter956/1
  UnitConverter956/1 -> VOUTP_FDCVMCDrInpTqBstGn_pct/1  "VOUTP_FDCVMCDrInpTqBstGn_pct"
